simulink model "SIM_EXO_DAL"  (R2021b)
(part 14 of 25)

t5537 = t7.*t9.*t34.*t191.*t200.*2.245376163391997e-22;
t5541 = -t5527;
t5542 = t34.*t191.*t199.*1.213683123456844e-22;
t5543 = t8.*t19.*t34.*t191.*t201.*1.598755564896737e-22;
t5544 = t8.*t9.*t34.*t191.*t201.*8.501479316957259e-23;
t5548 = -t5534;
t5550 = t5.*t8.*t9.*t34.*t191.*t201.*2.432291264259161e-22;
t5551 = t5.*t34.*t191.*t200.*3.069039723904487e-29;
t5553 = t5.*t7.*t9.*t34.*t191.*t200.*4.590123554345229e-22;
t5554 = t7.*t19.*t34.*t191.*t200.*6.983254769046087e-22;
t5556 = t5.*t7.*t34.*t191.*t200.*1.220412967321392e-22;
t5567 = -t5559;
t5568 = t7.*t34.*t191.*t200.*3.484557373753613e-22;
t5570 = t5.*t7.*t34.*t191.*t199.*8.811397961779761e-29;
t5571 = t9.*t34.*t191.*t200.*4.024651742608185e-29;
t5572 = t8.*t34.*t191.*t201.*5.756958141897304e-23;
t5585 = t7.*t9.*t34.*t191.*t199.*1.155501764459885e-28;
t5587 = t34.*t191.*t200.*7.426504311526687e-22;
t5588 = t34.*t191.*t201.*7.426504311526687e-22;
t5595 = -t5594;
t5598 = t2449+t2464;
t5599 = t3.*t5597;
t5601 = (t615.*t4119)./2.0;
t5608 = t5.*t34.*t191.*t202.*7.477660125089319e-22;
t5609 = -t5606;
t5610 = t9.*t34.*t191.*t202.*4.064278195638759e-22;
t5613 = -t5611;
t5614 = t34.*t191.*t202.*5.900961483070041e-22;
t5616 = t633+t636+t1432;
t5620 = t635+t637+t1430;
t5621 = (t4.*t640.*t4119)./2.0;
t5631 = t34.*t191.*t201.*7.59040540289635e-22;
t5636 = t1492+t4150;
t5658 = t199+t2422+t2472;
t5659 = t3230+t3242;
t5663 = t3243+t3256;
t5664 = t3.*t5656;
t5665 = t7.*t5656;
t5669 = t4.*t5660;
t5670 = t8.*t5660;
t5778 = t656+t2601+t3257;
t5781 = t655+t2600+t3276;
t5796 = t2550+t5600;
t5812 = t1467+t5667;
t5815 = t1474+t5668;
t5825 = dq4.*t5823;
t5917 = (t4119.*t5779)./2.0;
t5958 = (t4119.*t5826)./2.0;
t5998 = (t4.*t4119.*t5887)./2.0;
t5999 = (t8.*t4119.*t5886)./2.0;
t7149 = dq3.*t7148;
t214 = -t208;
t217 = -t212;
t661 = t9.*t646;
t677 = t5.*t646;
t729 = -t691;
t803 = -t740;
t848 = t18.*t680;
t850 = t23.*t680;
t893 = -t844;
t894 = -t845;
t905 = -t856;
t907 = -t859;
t908 = -t858;
t912 = -t865;
t913 = -t866;
t915 = -t867;
t919 = -t876;
t931 = t18.*t799;
t932 = t8.*t847;
t938 = t23.*t799;
t985 = -t943;
t990 = -t947;
t998 = t8.*t909;
t1031 = -t963;
t1088 = -t1017;
t1090 = -t1021;
t1156 = -t1072;
t1201 = -t1135;
t1212 = -t1145;
t1213 = -t1149;
t1289 = -t1237;
t1292 = -t1241;
t1502 = -t1491;
t1516 = -t1500;
t1525 = -t1509;
t1544 = t5.*t1509;
t1546 = t9.*t1509;
t1600 = -t1564;
t1628 = -t1579;
t1655 = -t1601;
t1656 = -t1602;
t1707 = t8.*t1583;
t1708 = t8.*t1585;
t1732 = t18.*t1526;
t1742 = t23.*t1526;
t1762 = -t1686;
t1821 = -t1721;
t1860 = t8.*t1675;
t1863 = -t1747;
t1868 = -t1753;
t1870 = t8.*t1691;
t1878 = t8.*t1700;
t1899 = t8.*t1715;
t1901 = -t1794;
t1922 = t18.*t1577;
t1929 = t23.*t1577;
t1940 = -t1846;
t1941 = -t1845;
t1974 = t8.*t1765;
t1990 = t8.*t1777;
t2010 = -t1902;
t2034 = t8.*t1845;
t2039 = -t1934;
t2145 = -t2049;
t2233 = -t2161;
t2234 = -t2160;
t2242 = -t2164;
t2297 = -t2260;
t2298 = -t2259;
t2299 = -t2261;
t2300 = -t2262;
t2328 = -t2293;
t2330 = -t2301;
t2332 = -t2303;
t2354 = -t2320;
t2473 = -t2465;
t2670 = -t2632;
t2679 = -t2643;
t2690 = t5.*t2622;
t2691 = t5.*t2623;
t2696 = t9.*t2622;
t2697 = t9.*t2623;
t2698 = t5.*t2628;
t2700 = t9.*t2628;
t2701 = t5.*t2632;
t2704 = t9.*t2632;
t2709 = t5.*t2647;
t2710 = t5.*t2648;
t2711 = t5.*t2649;
t2712 = t9.*t2647;
t2713 = t9.*t2648;
t2714 = t9.*t2649;
t2715 = t5.*t2613;
t2718 = t9.*t2613;
t2727 = t5.*t2660;
t2728 = t5.*t2661;
t2730 = t9.*t2660;
t2731 = t9.*t2661;
t2732 = t5.*t2664;
t2735 = t9.*t2664;
t2777 = -t2745;
t2779 = t5.*t2689;
t2794 = t5.*t2740;
t2813 = t5.*t2750;
t2836 = -t2790;
t2850 = -t2811;
t2851 = -t2810;
t2858 = t9.*t2780;
t2873 = t9.*t2785;
t2880 = -t2838;
t2881 = -t2837;
t2887 = -t2841;
t2889 = -t2843;
t2890 = t9.*t2807;
t2905 = -t2860;
t2906 = -t2859;
t2909 = -t2865;
t2912 = -t2871;
t2913 = -t2870;
t2915 = -t2875;
t2916 = -t2874;
t2917 = -t2876;
t2933 = -t2891;
t2987 = -t2934;
t2998 = -t2955;
t2999 = -t2954;
t3000 = -t2957;
t3015 = -t2974;
t3125 = -t3102;
t3129 = -t3107;
t3159 = -t3135;
t3161 = -t3136;
t3164 = -t3138;
t3166 = -t3141;
t3168 = -t3144;
t3220 = -t3201;
t3221 = -t3203;
t3222 = -t3202;
t3223 = -t3205;
t3224 = -t3204;
t3237 = -t3214;
t3238 = -t3216;
t3239 = -t3215;
t3246 = -t3226;
t3248 = -t3227;
t3266 = -t3235;
t3268 = -t3249;
t3591 = -t3561;
t3621 = t9.*t3565;
t3627 = -t3594;
t3628 = -t3595;
t3665 = t5.*t3588;
t3672 = t9.*t3561;
t3673 = t5.*t3565;
t3675 = t5.*t3566;
t3683 = -t3623;
t3684 = -t3626;
t3689 = -t3632;
t3764 = t9.*t3632;
t3765 = t5.*t3640;
t3767 = -t3685;
t3771 = t9.*t3640;
t3799 = -t3731;
t3807 = -t3739;
t3808 = -t3740;
t3809 = -t3741;
t3829 = t5.*t3623;
t3830 = t5.*t3624;
t3838 = t5.*t3698;
t3841 = t9.*t3698;
t3842 = t5.*t3703;
t3844 = -t3775;
t3848 = t9.*t3703;
t3859 = -t3719;
t3864 = t5.*t3727;
t3874 = t9.*t3731;
t3876 = t5.*t3742;
t3878 = t9.*t3742;
t3879 = -t3801;
t3880 = -t3802;
t3896 = -t3828;
t3900 = t9.*t3775;
t3904 = t5.*t3779;
t3905 = -t3837;
t3906 = t5.*t3781;
t3907 = t9.*t3781;
t3909 = t9.*t3782;
t3919 = -t3791;
t3920 = -t3856;
t3926 = -t3860;
t3927 = -t3861;
t3933 = t9.*t3801;
t3936 = t9.*t3802;
t3940 = t5.*t3812;
t3943 = t5.*t3818;
t3944 = t9.*t3818;
t3948 = -t3887;
t3955 = -t3902;
t3956 = -t3901;
t3957 = -t3903;
t3961 = t9.*t3856;
t3965 = t5.*t3865;
t3967 = t5.*t3868;
t3969 = t9.*t3868;
t3973 = -t3932;
t3975 = -t3935;
t3976 = -t3934;
t3977 = -t3938;
t3978 = -t3937;
t3979 = -t3939;
C_dq = ft_11({dq1,dq2,dq3,dq4,dq5,dq6,t1004,t1006,t1008,t1013,t1016,t1019,t1020,t1023,t1024,t1025,t1026,t1028,t1030,t1031,t1032,t1034,t1036,t1038,t1039,t1040,t1042,t1043,t1044,t1045,t1046,t1047,t1048,t1049,t1050,t1051,t1054,t1055,t1056,t1057,t1059,t1061,t1065,t1066,t1068,t1069,t1070,t1073,t1075,t1076,t1077,t1081,t1083,t1084,t1085,t1087,t1088,t1089,t1090,t1091,t1092,t1093,t1095,t1098,t1099,t1101,t1102,t1105,t1106,t1107,t1108,t1109,t111,t1113,t1115,t1116,t1119,t112,t1122,t1125,t1126,t1127,t1128,t113,t1130,t1131,t1133,t1134,t1138,t1139,t114,t1141,t1144,t1146,t1147,t1148,t115,t1150,t1152,t1153,t1155,t1156,t1158,t1159,t116,t1162,t1163,t1165,t1167,t1169,t1170,t1171,t1173,t1174,t1175,t1177,t1178,t1179,t1180,t1181,t1182,t1183,t1184,t1185,t1186,t1188,t1189,t1190,t1191,t1192,t1193,t1194,t1196,t1197,t1198,t1199,t1200,t1201,t1202,t1203,t1204,t1205,t1206,t1207,t121,t1210,t1211,t1212,t1213,t1215,t1219,t1221,t1222,t1224,t1225,t1227,t1228,t1233,t1235,t1236,t1239,t1240,t1244,t1245,t125,t1250,t1251,t1253,t1254,t1256,t1257,t1258,t1259,t126,t1261,t1262,t1263,t1264,t1265,t1266,t1267,t1268,t1269,t1271,t1272,t1273,t1274,t1277,t1278,t128,t1280,t1282,t1285,t1286,t1288,t1289,t1290,t1292,t1294,t1295,t1296,t1298,t1300,t1301,t1302,t1306,t1307,t1308,t1309,t131,t1311,t1312,t1313,t1315,t1316,t1317,t1318,t1319,t132,t1322,t1323,t1324,t1325,t1326,t1328,t1329,t133,t1330,t1331,t1333,t1337,t1338,t1340,t1341,t1342,t1343,t1344,t1345,t1346,t1348,t1351,t1352,t1353,t1354,t1355,t1356,t1360,t1362,t1365,t1366,t1367,t1369,t1370,t1371,t1372,t1374,t1375,t1377,t1378,t1379,t1380,t1383,t1384,t1385,t1386,t1388,t1389,t139,t1391,t1392,t1393,t1394,t1397,t140,t1401,t1402,t1403,t1404,t1406,t1407,t1408,t1409,t141,t1410,t1411,t1413,t1414,t1415,t1416,t1417,t1419,t142,t1423,t1426,t1427,t1428,t1429,t1431,t1433,t1436,t144,t1440,t1441,t1442,t1443,t1445,t1446,t1447,t1448,t1449,t1451,t1452,t1453,t1454,t1455,t1456,t1457,t1458,t1459,t1460,t1463,t1464,t1465,t1470,t1471,t1476,t1478,t1479,t148,t1481,t1482,t1483,t1486,t1487,t1488,t1489,t1490,t1493,t1494,t1495,t1496,t1498,t1499,t15,t150,t1501,t1502,t1503,t1505,t1506,t1507,t1508,t151,t1510,t1511,t1512,t1513,t1515,t1516,t1517,t1520,t1521,t1522,t1523,t1524,t1525,t1526,t1527,t1529,t153,t1530,t1531,t1532,t1533,t1534,t1535,t1536,t1537,t1538,t1539,t154,t1540,t1541,t1542,t1546,t1548,t1549,t1550,t1551,t1553,t1558,t156,t1560,t1561,t1562,t1566,t1567,t1568,t1570,t1571,t1572,t1574,t1575,t1576,t1577,t1578,t158,t1580,t1581,t1582,t1583,t1584,t1585,t1586,t1587,t1589,t1590,t1591,t1592,t1593,t1594,t1595,t1596,t1597,t1598,t1599,t16,t1600,t1601,t1602,t1605,t1606,t1607,t1609,t1610,t1611,t1612,t1613,t1614,t1615,t1616,t1617,t1618,t1619,t1620,t1621,t1622,t1625,t1626,t1627,t1628,t1630,t1631,t1632,t1633,t1635,t1636,t1637,t1638,t1639,t1641,t1642,t1643,t1644,t1645,t1646,t1647,t1648,t1651,t1652,t1653,t1655,t1656,t1657,t1658,t1659,t166,t1660,t1661,t1662,t1663,t1666,t1667,t1669,t1670,t1671,t1672,t1673,t1674,t1675,t1676,t1681,t1682,t1683,t1687,t1689,t1692,t1696,t1697,t1698,t1699,t17,t1700,t1701,t1702,t1703,t1704,t1705,t1706,t1707,t1708,t1709,t171,t1710,t1711,t1712,t1713,t1715,t1716,t1718,t1719,t1720,t1721,t1722,t1723,t1724,t1726,t1728,t1729,t1731,t1732,t1733,t1734,t1735,t1736,t1737,t1738,t1739,t1740,t1741,t1742,t1745,t1746,t1747,t1748,t1749,t1752,t1753,t1754,t1755,t1756,t1757,t1758,t1759,t1760,t1761,t1762,t1763,t1764,t1765,t1766,t1767,t1768,t1769,t1770,t1771,t1772,t1774,t1775,t1776,t1777,t1779,t1780,t1781,t1783,t1784,t1785,t1786,t1787,t1788,t1789,t1790,t1791,t1792,t1793,t1794,t1795,t1797,t1798,t1799,t18,t1800,t1801,t1804,t1805,t1806,t1807,t1808,t1809,t1810,t1811,t1812,t1813,t1814,t1815,t1816,t1817,t1820,t1821,t1822,t1823,t1824,t1827,t1828,t1829,t183,t1830,t1831,t1832,t1833,t1834,t1835,t1836,t1837,t1838,t1839,t1844,t1847,t1848,t1849,t185,t1850,t1851,t1853,t1855,t1856,t1857,t1858,t1859,t1860,t1861,t1863,t1864,t1865,t1866,t1867,t1868,t1870,t1871,t1873,t1877,t1878,t1879,t1881,t1882,t1884,t1885,t1886,t1887,t1889,t1891,t1892,t1893,t1896,t1899,t19,t190,t1900,t1901,t1902,t1903,t1905,t1906,t1907,t1908,t1909,t191,t1910,t1911,t1912,t1913,t1914,t1915,t1916,t1917,t1918,t1919,t1920,t1921,t1922,t1925,t1926,t1927,t1928,t1929,t1930,t1935,t1936,t1937,t1938,t1939,t1940,t1941,t1942,t1943,t1944,t1946,t1947,t1950,t1951,t1952,t1953,t1954,t1955,t196,t1961,t1966,t1967,t1968,t1969,t197,t1970,t1971,t1974,t1975,t1976,t1977,t1978,t1979,t1980,t1981,t1983,t1984,t1985,t1986,t1987,t1988,t1989,t199,t1990,t1991,t1992,t1993,t1994,t1995,t1996,t1997,t1998,t1999,t2,t20,t200,t2000,t2001,t2002,t2003,t2004,t2005,t2006,t2008,t201,t2010,t2011,t2014,t2015,t2016,t2017,t2018,t2019,t202,t2020,t2023,t2024,t2026,t2027,t2028,t2029,t203,t2033,t2034,t2035,t2036,t2037,t2038,t2039,t204,t2040,t2042,t2043,t2045,t2047,t205,t2050,t2051,t2052,t2053,t2054,t2056,t2057,t2058,t2059,t206,t2060,t2061,t2062,t2065,t2066,t2067,t2068,t2069,t207,t2070,t2071,t2072,t2073,t2074,t2075,t2076,t2077,t2078,t2079,t2081,t2082,t2083,t2084,t2085,t2086,t2087,t2088,t2089,t209,t2090,t2091,t2092,t2093,t2094,t2095,t2096,t2097,t2098,t2099,t21,t210,t2100,t2101,t2104,t2105,t2106,t2107,t2108,t2109,t211,t2110,t2111,t2113,t2114,t2115,t2116,t2117,t2118,t2119,t2121,t2123,t2125,t2127,t2128,t2129,t213,t2130,t2131,t2132,t2133,t2134,t2135,t2136,t2137,t2138,t214,t2142,t2143,t2144,t2145,t2146,t2148,t2149,t2150,t2151,t2152,t2154,t2155,t2156,t2157,t2158,t2159,t2164,t2165,t2166,t2169,t217,t2170,t2171,t2172,t2174,t2175,t2176,t2177,t2178,t2180,t2181,t2182,t2184,t2185,t2186,t2187,t2189,t2190,t2191,t2192,t2193,t2194,t2196,t2197,t2198,t2199,t22,t2200,t2201,t2202,t2203,t2204,t2208,t2209,t2211,t2212,t2213,t2214,t2215,t2216,t2217,t2218,t2219,t2220,t2221,t2223,t2224,t2225,t2227,t2228,t2229,t2230,t2231,t2232,t2233,t2234,t2236,t2237,t2238,t2239,t224,t2240,t2241,t2242,t2243,t2246,t2247,t2248,t2249,t225,t2251,t2253,t2254,t2256,t2257,t2258,t2263,t2264,t2265,t2266,t2267,t2268,t2269,t227,t2270,t2271,t2272,t2273,t2274,t2276,t2277,t2278,t2279,t228,t2280,t2281,t2282,t2283,t2284,t2285,t2286,t2288,t2289,t2290,t2291,t2295,t2296,t2297,t2298,t2299,t23,t230,t2300,t2302,t2303,t2304,t2305,t2306,t2307,t2308,t231,t2310,t2311,t2312,t2313,t2314,t2315,t2316,t2317,t2318,t2319,t2320,t2321,t2322,t2323,t2324,t2326,t2327,t2328,t233,t2330,t2331,t2332,t2333,t2334,t2336,t2337,t2338,t2339,t234,t2340,t2341,t2342,t2344,t2345,t2346,t2347,t2348,t235,t2350,t2354,t2355,t2357,t2358,t2359,t236,t2361,t2362,t2363,t2364,t2365,t2366,t2367,t2369,t2370,t2371,t2372,t2373,t2374,t2375,t2376,t2377,t2378,t2379,t2382,t2383,t2384,t2385,t2386,t2387,t2388,t2389,t2390,t2391,t2392,t2393,t2394,t2395,t2396,t2397,t2398,t24,t240,t2400,t2401,t2402,t2403,t2404,t2405,t2406,t2407,t2408,t2410,t2416,t2417,t2420,t2421,t2422,t2424,t2425,t2426,t2427,t2428,t2429,t243,t2430,t2431,t2434,t2435,t2437,t2438,t2439,t244,t2440,t2441,t2443,t2444,t2446,t2448,t2449,t2452,t2453,t2454,t2455,t2456,t2457,t2458,t2460,t2463,t2465,t2466,t2467,t2470,t2473,t2474,t2477,t2478,t2479,t2481,t2483,t2484,t2485,t2486,t2487,t2489,t249,t2490,t2494,t2495,t2497,t2500,t2502,t2503,t2505,t2507,t2508,t2510,t2511,t2512,t2513,t2517,t2518,t2519,t2520,t2521,t2522,t2523,t2524,t2525,t2526,t2527,t2530,t2531,t2533,t2534,t2535,t2536,t2537,t2539,t2540,t2541,t2542,t2543,t2544,t2545,t2546,t2547,t2548,t2549,t2552,t2553,t2554,t2555,t2556,t2560,t2562,t2563,t2564,t2565,t2566,t2567,t2568,t2569,t257,t2570,t2571,t2574,t2575,t2576,t2577,t2578,t2579,t258,t2581,t2582,t2585,t2586,t2587,t2588,t2589,t2590,t2594,t2595,t2597,t2598,t2599,t2602,t2603,t2604,t2606,t2607,t2608,t2611,t2612,t2613,t2614,t2615,t2616,t2617,t2620,t2622,t2623,t2624,t2625,t2626,t2627,t2628,t2629,t263,t2630,t2631,t2633,t2634,t2636,t2639,t2640,t2641,t2644,t2647,t2648,t2649,t2650,t2651,t2654,t2655,t2656,t2657,t2659,t266,t2660,t2661,t2662,t2663,t2664,t2665,t2666,t2668,t2669,t2670,t2671,t2673,t2675,t2676,t2677,t2678,t2679,t2680,t2681,t2682,t2684,t2685,t2686,t2688,t2689,t2691,t2692,t2693,t2694,t2695,t2696,t2697,t2698,t2699,t270,t2700,t2701,t2705,t2706,t2707,t2708,t2711,t2712,t2713,t2714,t2715,t2718,t2719,t2720,t2721,t2722,t2723,t2724,t2725,t2726,t2728,t2729,t273,t2730,t2731,t2732,t2735,t2736,t2737,t2738,t274,t2740,t2741,t2742,t2743,t2744,t2746,t2747,t2748,t2749,t275,t2750,t2752,t2753,t2754,t2755,t2756,t2757,t2758,t2759,t276,t2760,t2761,t2762,t2763,t2764,t2765,t2766,t2767,t2769,t277,t2770,t2771,t2772,t2774,t2775,t2777,t2778,t278,t2780,t2783,t2784,t2785,t2791,t2792,t2793,t2795,t2796,t2797,t2798,t2799,t280,t2800,t2801,t2802,t2803,t2805,t2806,t2807,t2809,t2812,t2814,t2815,t2816,t2817,t2818,t2819,t2820,t2822,t2823,t2824,t2825,t2826,t2827,t2828,t2829,t2830,t2831,t2832,t2833,t2834,t2835,t2836,t2839,t284,t2842,t2844,t2845,t2846,t2850,t2851,t2852,t2854,t2857,t2861,t2863,t2864,t2867,t2868,t2869,t287,t2872,t2877,t2878,t2880,t2881,t2882,t2883,t2884,t2885,t2886,t2887,t2888,t2889,t2892,t2893,t2894,t2895,t2896,t2897,t29,t290,t2900,t2903,t2904,t2905,t2906,t2907,t2908,t2909,t291,t2910,t2911,t2912,t2913,t2914,t2915,t2916,t2917,t2918,t2919,t292,t2920,t2921,t2922,t2923,t2925,t2928,t2929,t2930,t2931,t2932,t2933,t2937,t294,t2940,t2941,t2942,t2944,t2945,t2946,t2947,t2949,t2950,t2951,t2952,t2956,t2958,t2959,t2962,t2965,t2966,t2967,t2968,t2969,t297,t2970,t2971,t2972,t2973,t2975,t2977,t2978,t2980,t2983,t2984,t2985,t2986,t2987,t2988,t2989,t299,t2991,t2992,t2993,t2994,t2995,t2996,t2997,t2998,t2999,t3,t30,t300,t3000,t3001,t3002,t3003,t3005,t3007,t3008,t3010,t3011,t3013,t3014,t3015,t3018,t3019,t302,t3020,t3021,t3022,t3024,t3025,t3027,t3029,t303,t3030,t3031,t3032,t3033,t3034,t3035,t3036,t3037,t3038,t304,t3041,t3043,t3044,t3046,t3047,t3048,t3049,t305,t3050,t3051,t3052,t3053,t3054,t3055,t3056,t3057,t3059,t306,t3060,t3061,t3062,t3064,t3065,t3066,t3067,t3068,t3069,t3070,t3071,t3072,t3073,t3074,t3076,t3077,t3079,t3080,t3081,t3082,t3083,t3084,t3085,t3086,t3088,t3089,t309,t3090,t3092,t3094,t3095,t3096,t3097,t3098,t3099,t310,t3100,t3103,t3104,t3105,t3106,t3108,t3109,t311,t3110,t3112,t3113,t3114,t3117,t3118,t3119,t3120,t3121,t3122,t3123,t3124,t3125,t3126,t3127,t3128,t3129,t313,t3130,t3131,t3132,t3133,t3134,t3136,t3139,t314,t3140,t3142,t3143,t3146,t3148,t3149,t315,t3150,t3152,t3153,t3154,t3156,t3157,t3158,t3159,t316,t3160,t3161,t3163,t3164,t3166,t3167,t3168,t3169,t3170,t3171,t3172,t3174,t3175,t3176,t3178,t3179,t318,t3180,t3182,t3183,t3184,t3185,t3186,t3187,t3188,t3189,t319,t3190,t3191,t3192,t3193,t3194,t3195,t3196,t3198,t3199,t320,t3200,t3207,t3208,t3209,t3210,t3213,t3217,t3219,t322,t3220,t3221,t3222,t3223,t3224,t3228,t3229,t3230,t3232,t3234,t3236,t3237,t3238,t3239,t324,t3240,t3245,t3246,t3247,t3248,t325,t3250,t3251,t3252,t3254,t3265,t3266,t3267,t3268,t3269,t3270,t3271,t3272,t3273,t3274,t3275,t3277,t3278,t3279,t328,t3280,t3282,t3283,t3284,t3285,t3286,t3287,t3288,t3289,t3290,t3291,t3292,t3293,t3295,t3296,t3297,t3298,t3299,t3301,t3302,t3303,t3306,t3307,t3308,t3309,t3310,t3312,t3313,t3314,t3317,t3318,t3320,t3321,t3322,t3323,t3324,t3325,t3326,t3327,t3328,t3329,t333,t3331,t3332,t3333,t3334,t3335,t3336,t3337,t3338,t3339,t3340,t3341,t3342,t3343,t3346,t3347,t3349,t3350,t3351,t3352,t3353,t3354,t3356,t3357,t3358,t3359,t336,t3360,t3362,t3363,t3364,t3365,t3366,t3367,t3368,t3369,t337,t3371,t3372,t3373,t3374,t3375,t3376,t3377,t3378,t3380,t3381,t3382,t3383,t3384,t3386,t3387,t3388,t3390,t3391,t3392,t3393,t3394,t3395,t3396,t3397,t3398,t3399,t34,t340,t3400,t3402,t3403,t3404,t3405,t3407,t3408,t3409,t3410,t3411,t3412,t3413,t3416,t3417,t3418,t3420,t3421,t3422,t3423,t3424,t3425,t3426,t3427,t3429,t3430,t3431,t3432,t3433,t3434,t3435,t3436,t3437,t3439,t344,t3440,t3441,t3442,t3443,t3444,t3445,t3446,t3447,t3448,t3449,t3450,t3453,t3454,t3455,t3456,t3457,t3458,t346,t3460,t3461,t3462,t3463,t3464,t3465,t3466,t3467,t3468,t3469,t347,t3470,t3471,t3472,t3473,t3474,t3475,t3476,t3479,t348,t3480,t3481,t3483,t3484,t3485,t3487,t3488,t3489,t349,t3490,t3491,t3492,t3493,t3494,t3496,t3497,t3498,t3499,t350,t3500,t3501,t3502,t3503,t3504,t3505,t3506,t3507,t3509,t3510,t3511,t3513,t3514,t3515,t3516,t3517,t3518,t352,t3521,t3522,t3523,t3526,t3529,t353,t3530,t3531,t3532,t3533,t3535,t3536,t3538,t3539,t3540,t3542,t3543,t3544,t3546,t3547,t3549,t3551,t3552,t3554,t3556,t3557,t3559,t356,t3560,t3562,t3563,t3564,t3565,t3566,t3568,t3569,t357,t3570,t3571,t3572,t3573,t3574,t3577,t3578,t358,t3582,t3583,t3584,t3585,t3586,t3587,t3588,t3589,t359,t3590,t3591,t3592,t3593,t3595,t3596,t3597,t3598,t3599,t3600,t3602,t3603,t3604,t3605,t3606,t3607,t3609,t361,t3610,t3611,t3612,t3616,t3617,t3618,t362,t3624,t3625,t3627,t3628,t3630,t3631,t3633,t3634,t3635,t3636,t3637,t3638,t3640,t3642,t3644,t3648,t365,t3652,t3653,t3654,t3655,t3656,t3657,t3658,t3659,t3660,t3662,t3663,t3664,t3665,t3666,t3667,t3668,t3669,t3670,t3671,t3672,t3673,t3674,t3675,t3676,t3677,t3678,t3679,t368,t3681,t3682,t3683,t3684,t3687,t3689,t369,t3690,t3691,t3692,t3693,t3694,t3695,t3696,t3697,t3698,t3699,t3700,t3701,t3702,t3703,t3704,t3705,t3706,t3707,t3708,t3709,t371,t3711,t3712,t3713,t3715,t3716,t3717,t3718,t3719,t372,t3720,t3724,t3725,t3726,t3727,t3728,t3729,t373,t3730,t3731,t3732,t3733,t3734,t3735,t3736,t3737,t3738,t374,t3740,t3742,t3743,t3744,t3745,t3746,t3747,t3750,t3752,t3753,t3754,t3755,t3756,t3757,t3758,t3759,t3760,t3761,t3762,t3763,t3764,t3765,t3766,t3767,t3768,t3769,t377,t3772,t3774,t3777,t3778,t3779,t378,t3780,t3781,t3782,t3783,t3784,t3785,t3786,t3787,t3788,t3789,t379,t3790,t3791,t3792,t3793,t3794,t3795,t3796,t3797,t3798,t3799,t380,t3800,t3807,t3808,t3809,t3810,t3811,t3812,t3813,t3814,t3815,t3816,t3817,t3818,t3819,t382,t3820,t3821,t3822,t3823,t3824,t3825,t3830,t3831,t3833,t3834,t3835,t3836,t3838,t3839,t384,t3840,t3841,t3842,t3843,t3844,t3845,t3848,t3849,t3850,t3851,t3852,t3853,t3855,t3859,t386,t3861,t3862,t3863,t3864,t3865,t3866,t3868,t3869,t387,t3870,t3871,t3872,t3873,t3874,t3875,t3876,t3877,t3879,t388,t3880,t3881,t3882,t3883,t3884,t3885,t3886,t3888,t3889,t3890,t3891,t3892,t3893,t3894,t3895,t3896,t3897,t3899,t3900,t3904,t3905,t3906,t3907,t3908,t3909,t391,t3910,t3911,t3912,t3913,t3914,t3915,t3916,t3917,t3918,t3919,t392,t3920,t3921,t3922,t3923,t3924,t3925,t3926,t3927,t3928,t3931,t3936,t3940,t3941,t3942,t3943,t3944,t3946,t3948,t395,t3950,t3951,t3952,t3953,t3954,t3955,t3956,t3957,t3958,t3959,t396,t3960,t3961,t3962,t3963,t3964,t3965,t3966,t3967,t3968,t3969,t3971,t3972,t3973,t3974,t3975,t3976,t3977,t3978,t3979,t3982,t3983,t3984,t3985,t3986,t3987,t3988,t3989,t3994,t3995,t3996,t3997,t4,t400,t4000,t4003,t4004,t4006,t4008,t4009,t401,t4010,t4011,t4012,t4013,t4014,t4015,t4016,t4017,t4018,t4019,t402,t4020,t4022,t4023,t4024,t4025,t4026,t4028,t4029,t403,t4034,t4035,t4037,t4038,t4039,t4040,t4041,t4042,t4045,t4046,t4047,t4048,t4049,t4050,t4051,t4053,t4054,t4055,t4056,t4057,t4059,t406,t4060,t4061,t4062,t4063,t4064,t4065,t4066,t4067,t4068,t4069,t4070,t4071,t4073,t4074,t4075,t4079,t4080,t4081,t4082,t4083,t4084,t4085,t4086,t4087,t4089,t4090,t4091,t4092,t4093,t4094,t4095,t4097,t4098,t4099,t410,t4100,t4103,t4105,t4106,t4108,t4109,t411,t4110,t4111,t4112,t4113,t4114,t4115,t4116,t4118,t4119,t412,t4120,t4123,t4124,t4125,t4126,t4127,t4128,t4129,t413,t4130,t4132,t4133,t4134,t4135,t4136,t4139,t414,t4140,t4141,t4142,t4143,t4144,t4145,t4147,t4148,t4149,t415,t4151,t4152,t4153,t4154,t416,t4161,t4162,t4164,t4165,t4166,t4169,t417,t4171,t4173,t4174,t4177,t4178,t4179,t418,t4180,t4181,t4183,t4184,t4185,t4186,t4188,t4190,t4195,t4196,t4197,t420,t4201,t4202,t4205,t4206,t4207,t4208,t4209,t4210,t4211,t4215,t4217,t4218,t4219,t422,t4220,t4221,t4223,t4224,t4225,t4226,t4228,t4229,t423,t4230,t4231,t4232,t4233,t4234,t4235,t424,t4241,t4242,t4243,t4244,t4245,t4246,t4247,t4248,t4249,t425,t4250,t4251,t4253,t4254,t4255,t4256,t4257,t4258,t4259,t4260,t4261,t4262,t4263,t427,t4273,t4274,t4275,t4276,t4278,t4279,t428,t4280,t4281,t4282,t4283,t4284,t4285,t4286,t4287,t4289,t429,t4290,t4291,t4292,t4293,t4295,t4296,t4297,t4298,t4299,t4300,t4301,t4302,t4303,t4304,t4305,t4306,t4308,t431,t4310,t4315,t4316,t4317,t4318,t432,t4321,t4323,t4324,t4325,t4326,t4327,t4328,t4329,t433,t4330,t4331,t4332,t4333,t4334,t4335,t4336,t4337,t4338,t4339,t434,t4340,t4342,t4344,t4345,t4346,t4347,t4348,t4349,t435,t4350,t4354,t4356,t4357,t436,t4362,t4363,t4365,t4366,t4368,t4369,t437,t4370,t4371,t4372,t4373,t4374,t4375,t4376,t4377,t4378,t4379,t438,t4380,t4382,t4383,t4384,t4385,t4386,t4387,t4388,t4389,t439,t4391,t4392,t4394,t4395,t4396,t4397,t4398,t4399,t44,t440,t4400,t4401,t4402,t4403,t4404,t4405,t4406,t4407,t4408,t4409,t441,t4410,t4411,t4412,t4413,t4414,t4415,t4416,t4417,t4418,t4419,t442,t4420,t4421,t4422,t4423,t4424,t4425,t4426,t4427,t4428,t4429,t4430,t4431,t4432,t4433,t4434,t4435,t4436,t4437,t4438,t4439,t444,t4440,t4442,t4444,t4445,t4446,t4447,t4448,t4449,t445,t4450,t4451,t4453,t4454,t4455,t4460,t4461,t4462,t4463,t4464,t4465,t4466,t4467,t4468,t4469,t4470,t4471,t4473,t4474,t4475,t4476,t4477,t4478,t4479,t448,t4481,t4482,t4483,t4484,t4485,t4486,t4487,t4488,t4489,t449,t4490,t4493,t4494,t4495,t4496,t4497,t4498,t4499,t45,t450,t4500,t4501,t4502,t4503,t4504,t4505,t4506,t4507,t4508,t4509,t4510,t4512,t4513,t4514,t4515,t4516,t4518,t4519,t452,t4520,t4521,t4522,t4523,t4524,t4525,t4526,t4527,t4529,t453,t4530,t4531,t4532,t4534,t4535,t4536,t4537,t4538,t4539,t454,t4541,t4543,t4544,t4545,t4546,t4547,t4549,t4550,t4551,t4552,t4553,t4554,t4556,t4557,t4558,t4559,t4560,t4564,t4565,t4566,t4567,t4568,t4569,t457,t4570,t4572,t4573,t4575,t4576,t4577,t4578,t458,t4580,t4581,t4582,t4584,t4585,t4586,t4587,t4588,t4589,t459,t4590,t4591,t4592,t4593,t4594,t4595,t4596,t4597,t4598,t4599,t46,t460,t4600,t4601,t4602,t4603,t4604,t4605,t4606,t4607,t4608,t4609,t461,t4610,t4612,t4613,t4614,t4615,t4616,t4617,t4618,t4619,t462,t4620,t4621,t4622,t4623,t4624,t4625,t4626,t4627,t4629,t463,t4631,t4632,t4633,t4634,t4635,t4636,t4637,t4638,t4639,t464,t4640,t4643,t4644,t4645,t4646,t4647,t4648,t4649,t465,t4650,t4652,t4653,t4654,t4655,t4656,t4657,t4659,t466,t4660,t4661,t4662,t4663,t4664,t4665,t4666,t4667,t4668,t4669,t4670,t4671,t4672,t4673,t4674,t4675,t4676,t4677,t4678,t4679,t468,t4680,t4681,t4682,t4683,t4684,t4685,t4686,t4687,t4689,t469,t4692,t4693,t4694,t4695,t4696,t4697,t4698,t4699,t47,t470,t4700,t4702,t4703,t4704,t4707,t4708,t4709,t471,t4710,t4711,t4712,t4713,t4714,t4715,t4716,t4717,t4718,t4719,t472,t4720,t4721,t4722,t4723,t4724,t4725,t4726,t4727,t4728,t4729,t4730,t4731,t4732,t4733,t4734,t4736,t4737,t4738,t4739,t4740,t4742,t4745,t4746,t4747,t4748,t475,t4750,t4751,t4753,t4754,t4755,t4756,t4757,t4762,t4763,t4765,t4768,t477,t4771,t4772,t4773,t4774,t4775,t4776,t4779,t4780,t4781,t4782,t4783,t4784,t4785,t4786,t4787,t4788,t4789,t479,t4790,t4791,t4792,t4793,t4794,t4795,t4797,t4799,t480,t4800,t4801,t4802,t4803,t4805,t4806,t4809,t481,t4810,t4811,t4812,t4813,t4814,t4816,t4817,t4818,t4819,t482,t4820,t4822,t4823,t4824,t4825,t4826,t4827,t4829,t483,t4831,t4833,t4834,t4835,t4837,t484,t4840,t4841,t4842,t4843,t4844,t4845,t4846,t4848,t485,t4850,t4853,t4854,t4855,t4856,t4857,t4858,t4859,t486,t4862,t4863,t4864,t4865,t4866,t4867,t4868,t4869,t4870,t4872,t4873,t4874,t4875,t4876,t4877,t488,t4880,t4881,t4884,t4888,t4889,t489,t4890,t4893,t4894,t4895,t4896,t4898,t4901,t4902,t4903,t4904,t4905,t4906,t4907,t4908,t491,t4911,t4913,t4914,t4919,t492,t4920,t4922,t4924,t4925,t4927,t4928,t4929,t493,t4931,t4932,t4933,t4934,t4935,t4936,t4939,t494,t4942,t4943,t4944,t4946,t4947,t4948,t4949,t4950,t4951,t4952,t4953,t4957,t4959,t496,t4960,t4961,t4963,t4964,t4965,t4966,t4967,t4969,t497,t4970,t4973,t4974,t4975,t4976,t4978,t4979,t498,t4981,t4982,t4983,t4984,t4987,t4988,t4989,t499,t4990,t4991,t4992,t4993,t4994,t4995,t4996,t5,t50,t500,t5000,t5001,t5002,t5003,t5005,t5006,t5007,t5008,t5009,t501,t5010,t5013,t5014,t5015,t5016,t5017,t5018,t5019,t502,t5020,t5021,t5022,t5023,t5024,t5026,t5027,t5028,t5029,t503,t5031,t5032,t5035,t5036,t5037,t5039,t504,t5041,t5045,t5047,t5048,t505,t5051,t5054,t5055,t5056,t5057,t5058,t5059,t506,t5061,t5063,t5064,t5065,t5066,t5067,t5068,t507,t5073,t5074,t5075,t5076,t5077,t5078,t5079,t508,t5080,t5083,t5084,t5085,t5086,t5087,t5088,t5089,t509,t5090,t5091,t5092,t5093,t5094,t5095,t5097,t5098,t5099,t510,t5100,t5101,t5102,t5103,t5104,t5105,t5107,t5109,t511,t5110,t5112,t5113,t5114,t5117,t5118,t5119,t512,t5120,t5121,t5123,t5124,t5126,t5128,t513,t5131,t5132,t5133,t5134,t5135,t5136,t5137,t5138,t5139,t514,t5140,t5141,t5143,t5146,t5147,t5148,t5150,t5151,t5154,t5156,t5157,t5158,t5159,t516,t5160,t5162,t5164,t5166,t5167,t517,t5171,t5172,t5173,t5174,t5175,t5177,t518,t5180,t5181,t5182,t5183,t5184,t5185,t5187,t5188,t5189,t5190,t5191,t5194,t5195,t5197,t5199,t520,t5200,t5201,t5202,t5203,t5204,t5205,t5206,t5207,t5209,t521,t5210,t5211,t5213,t5214,t5215,t5216,t5217,t5218,t5219,t522,t5220,t5221,t5222,t5223,t5224,t5225,t5226,t5227,t5229,t523,t5233,t5236,t5237,t5238,t5239,t524,t5240,t5242,t5243,t5244,t5247,t5248,t5249,t525,t5251,t5252,t5255,t5258,t526,t5261,t5262,t5265,t5268,t5269,t527,t5270,t5272,t5275,t5276,t5277,t5278,t5279,t528,t5280,t5285,t5287,t5288,t529,t5291,t5292,t5293,t5294,t5295,t5297,t5298,t53,t530,t5302,t5303,t5304,t5306,t5308,t531,t5310,t5317,t5318,t532,t5320,t5321,t5322,t5324,t5326,t5327,t5329,t533,t5330,t5331,t5332,t5334,t5336,t5339,t534,t5341,t5344,t5346,t5347,t5348,t5349,t535,t5351,t5355,t5356,t5358,t5359,t536,t5361,t5364,t5365,t5367,t5368,t537,t5372,t5373,t5374,t5375,t5378,t538,t5383,t5386,t5387,t5388,t5389,t539,t5390,t5391,t5392,t5393,t5394,t5395,t540,t5402,t5404,t5406,t5408,t5409,t5411,t5416,t5420,t543,t5433,t5435,t5436,t5437,t5438,t544,t5440,t5441,t5442,t5443,t5444,t5445,t5448,t545,t5450,t5451,t5453,t5454,t5457,t5459,t546,t5460,t5461,t5462,t5463,t5464,t5465,t5466,t547,t5473,t5475,t5479,t548,t5480,t5481,t5482,t5483,t5484,t5485,t5486,t5487,t5488,t5489,t549,t5490,t5491,t5492,t5493,t5494,t5495,t5498,t5499,t5500,t5501,t5502,t5503,t5504,t5505,t5506,t5507,t551,t5512,t5513,t5514,t5516,t5517,t5518,t5519,t552,t5520,t5521,t5523,t5524,t5525,t5526,t5528,t553,t5531,t5533,t5536,t5537,t554,t5540,t5541,t5542,t5543,t5544,t5546,t5548,t5549,t555,t5550,t5551,t5552,t5553,t5554,t5555,t5556,t556,t5561,t5562,t5563,t5565,t5566,t5567,t5568,t5569,t557,t5570,t5571,t5572,t5573,t5578,t558,t5580,t5581,t5583,t5584,t5585,t5587,t5588,t5589,t559,t5590,t5593,t5595,t5596,t5599,t560,t5601,t5603,t5604,t5607,t5608,t5609,t561,t5610,t5612,t5613,t5614,t5616,t5618,t562,t5620,t5621,t5629,t563,t5631,t5633,t5634,t5635,t5636,t564,t5658,t5664,t5665,t5669,t567,t5670,t5673,t5678,t568,t5688,t569,t57,t570,t571,t572,t573,t574,t5741,t5743,t576,t577,t5777,t5778,t5779,t578,t5780,t5781,t5782,t579,t58,t580,t581,t5815,t5818,t5819,t582,t5823,t5825,t5826,t583,t584,t586,t587,t5886,t5887,t589,t5894,t59,t590,t591,t5917,t592,t593,t594,t595,t5958,t596,t597,t5998,t5999,t6,t60,t600,t602,t603,t604,t605,t609,t610,t611,t612,t613,t614,t615,t616,t618,t619,t620,t621,t622,t623,t624,t625,t626,t629,t632,t633,t634,t638,t639,t640,t641,t642,t643,t645,t646,t647,t648,t649,t650,t653,t654,t657,t658,t660,t661,t662,t663,t664,t665,t667,t668,t669,t673,t674,t675,t676,t677,t679,t680,t681,t682,t683,t684,t685,t686,t687,t688,t689,t692,t693,t694,t695,t696,t697,t698,t7,t700,t702,t703,t704,t705,t706,t708,t71,t710,t711,t712,t713,t7148,t7149,t715,t716,t72,t724,t728,t729,t73,t731,t733,t734,t735,t736,t738,t739,t74,t741,t742,t743,t744,t746,t747,t748,t749,t75,t750,t751,t752,t753,t754,t755,t756,t757,t758,t759,t76,t760,t762,t763,t764,t765,t766,t767,t768,t769,t77,t772,t773,t774,t775,t776,t777,t778,t779,t780,t781,t782,t784,t785,t786,t792,t794,t795,t796,t797,t798,t799,t8,t80,t801,t802,t803,t804,t805,t806,t808,t81,t814,t815,t817,t820,t822,t823,t824,t825,t826,t827,t829,t83,t830,t831,t832,t833,t834,t835,t836,t837,t838,t84,t840,t841,t842,t843,t845,t846,t847,t848,t852,t853,t856,t86,t861,t863,t866,t868,t869,t870,t874,t875,t876,t877,t878,t880,t881,t882,t884,t885,t888,t891,t893,t894,t895,t899,t9,t90,t900,t902,t903,t905,t906,t907,t908,t909,t91,t910,t911,t912,t913,t914,t915,t916,t917,t919,t920,t921,t922,t923,t925,t926,t927,t928,t929,t930,t931,t932,t934,t935,t937,t940,t941,t942,t943,t944,t945,t946,t947,t949,t95,t950,t951,t952,t953,t954,t955,t957,t958,t961,t962,t964,t965,t968,t97,t970,t971,t972,t973,t974,t975,t976,t977,t982,t983,t984,t985,t986,t987,t988,t989,t99,t990,t991,t993,t994,t995,t998,t999});
end
function C_dq = ft_11(ct)
dq1 = ct{1};
dq2 = ct{2};
dq3 = ct{3};
dq4 = ct{4};
dq5 = ct{5};
dq6 = ct{6};
t1004 = ct{7};
t1006 = ct{8};
t1008 = ct{9};
t1013 = ct{10};
t1016 = ct{11};
t1019 = ct{12};
t1020 = ct{13};
t1023 = ct{14};
t1024 = ct{15};
t1025 = ct{16};
t1026 = ct{17};
t1028 = ct{18};
t1030 = ct{19};
t1031 = ct{20};
t1032 = ct{21};
t1034 = ct{22};
t1036 = ct{23};
t1038 = ct{24};
t1039 = ct{25};
t1040 = ct{26};
t1042 = ct{27};
t1043 = ct{28};
t1044 = ct{29};
t1045 = ct{30};
t1046 = ct{31};
t1047 = ct{32};
t1048 = ct{33};
t1049 = ct{34};
t1050 = ct{35};
t1051 = ct{36};
t1054 = ct{37};
t1055 = ct{38};
t1056 = ct{39};
t1057 = ct{40};
t1059 = ct{41};
t1061 = ct{42};
t1065 = ct{43};
t1066 = ct{44};
t1068 = ct{45};
t1069 = ct{46};
t1070 = ct{47};
t1073 = ct{48};
t1075 = ct{49};
t1076 = ct{50};
t1077 = ct{51};
t1081 = ct{52};
t1083 = ct{53};
t1084 = ct{54};
t1085 = ct{55};
t1087 = ct{56};
t1088 = ct{57};
t1089 = ct{58};
t1090 = ct{59};
t1091 = ct{60};
t1092 = ct{61};
t1093 = ct{62};
t1095 = ct{63};
t1098 = ct{64};
t1099 = ct{65};
t1101 = ct{66};
t1102 = ct{67};
t1105 = ct{68};
t1106 = ct{69};
t1107 = ct{70};
t1108 = ct{71};
t1109 = ct{72};
t111 = ct{73};
t1113 = ct{74};
t1115 = ct{75};
t1116 = ct{76};
t1119 = ct{77};
t112 = ct{78};
t1122 = ct{79};
t1125 = ct{80};
t1126 = ct{81};
t1127 = ct{82};
t1128 = ct{83};
t113 = ct{84};
t1130 = ct{85};
t1131 = ct{86};
t1133 = ct{87};
t1134 = ct{88};
t1138 = ct{89};
t1139 = ct{90};
t114 = ct{91};
t1141 = ct{92};
t1144 = ct{93};
t1146 = ct{94};
t1147 = ct{95};
t1148 = ct{96};
t115 = ct{97};
t1150 = ct{98};
t1152 = ct{99};
t1153 = ct{100};
t1155 = ct{101};
t1156 = ct{102};
t1158 = ct{103};
t1159 = ct{104};
t116 = ct{105};
t1162 = ct{106};
t1163 = ct{107};
t1165 = ct{108};
t1167 = ct{109};
t1169 = ct{110};
t1170 = ct{111};
t1171 = ct{112};
t1173 = ct{113};
t1174 = ct{114};
t1175 = ct{115};
t1177 = ct{116};
t1178 = ct{117};
t1179 = ct{118};
t1180 = ct{119};
t1181 = ct{120};
t1182 = ct{121};
t1183 = ct{122};
t1184 = ct{123};
t1185 = ct{124};
t1186 = ct{125};
t1188 = ct{126};
t1189 = ct{127};
t1190 = ct{128};
t1191 = ct{129};
t1192 = ct{130};
t1193 = ct{131};
t1194 = ct{132};
t1196 = ct{133};
t1197 = ct{134};
t1198 = ct{135};
t1199 = ct{136};
t1200 = ct{137};
t1201 = ct{138};
t1202 = ct{139};
t1203 = ct{140};
t1204 = ct{141};
t1205 = ct{142};
t1206 = ct{143};
t1207 = ct{144};
t121 = ct{145};
t1210 = ct{146};
t1211 = ct{147};
t1212 = ct{148};
t1213 = ct{149};
t1215 = ct{150};
t1219 = ct{151};
t1221 = ct{152};
t1222 = ct{153};
t1224 = ct{154};
t1225 = ct{155};
t1227 = ct{156};
t1228 = ct{157};
t1233 = ct{158};
t1235 = ct{159};
t1236 = ct{160};
t1239 = ct{161};
t1240 = ct{162};
t1244 = ct{163};
t1245 = ct{164};
t125 = ct{165};
t1250 = ct{166};
t1251 = ct{167};
t1253 = ct{168};
t1254 = ct{169};
t1256 = ct{170};
t1257 = ct{171};
t1258 = ct{172};
t1259 = ct{173};
t126 = ct{174};
t1261 = ct{175};
t1262 = ct{176};
t1263 = ct{177};
t1264 = ct{178};
t1265 = ct{179};
t1266 = ct{180};
t1267 = ct{181};
t1268 = ct{182};
t1269 = ct{183};
t1271 = ct{184};
t1272 = ct{185};
t1273 = ct{186};
t1274 = ct{187};
t1277 = ct{188};
t1278 = ct{189};
t128 = ct{190};
t1280 = ct{191};
t1282 = ct{192};
t1285 = ct{193};
t1286 = ct{194};
t1288 = ct{195};
t1289 = ct{196};
t1290 = ct{197};
t1292 = ct{198};
t1294 = ct{199};
t1295 = ct{200};
t1296 = ct{201};
t1298 = ct{202};
t1300 = ct{203};
t1301 = ct{204};
t1302 = ct{205};
t1306 = ct{206};
t1307 = ct{207};
t1308 = ct{208};
t1309 = ct{209};
t131 = ct{210};
t1311 = ct{211};
t1312 = ct{212};
t1313 = ct{213};
t1315 = ct{214};
t1316 = ct{215};
t1317 = ct{216};
t1318 = ct{217};
t1319 = ct{218};
t132 = ct{219};
t1322 = ct{220};
t1323 = ct{221};
t1324 = ct{222};
t1325 = ct{223};
t1326 = ct{224};
t1328 = ct{225};
t1329 = ct{226};
t133 = ct{227};
t1330 = ct{228};
t1331 = ct{229};
t1333 = ct{230};
t1337 = ct{231};
t1338 = ct{232};
t1340 = ct{233};
t1341 = ct{234};
t1342 = ct{235};
t1343 = ct{236};
t1344 = ct{237};
t1345 = ct{238};
t1346 = ct{239};
t1348 = ct{240};
t1351 = ct{241};
t1352 = ct{242};
t1353 = ct{243};
t1354 = ct{244};
t1355 = ct{245};
t1356 = ct{246};
t1360 = ct{247};
t1362 = ct{248};
t1365 = ct{249};
t1366 = ct{250};
t1367 = ct{251};
t1369 = ct{252};
t1370 = ct{253};
t1371 = ct{254};
t1372 = ct{255};
t1374 = ct{256};
t1375 = ct{257};
t1377 = ct{258};
t1378 = ct{259};
t1379 = ct{260};
t1380 = ct{261};
t1383 = ct{262};
t1384 = ct{263};
t1385 = ct{264};
t1386 = ct{265};
t1388 = ct{266};
t1389 = ct{267};
t139 = ct{268};
t1391 = ct{269};
t1392 = ct{270};
t1393 = ct{271};
t1394 = ct{272};
t1397 = ct{273};
t140 = ct{274};
t1401 = ct{275};
t1402 = ct{276};
t1403 = ct{277};
t1404 = ct{278};
t1406 = ct{279};
t1407 = ct{280};
t1408 = ct{281};
t1409 = ct{282};
t141 = ct{283};
t1410 = ct{284};
t1411 = ct{285};
t1413 = ct{286};
t1414 = ct{287};
t1415 = ct{288};
t1416 = ct{289};
t1417 = ct{290};
t1419 = ct{291};
t142 = ct{292};
t1423 = ct{293};
t1426 = ct{294};
t1427 = ct{295};
t1428 = ct{296};
t1429 = ct{297};
t1431 = ct{298};
t1433 = ct{299};
t1436 = ct{300};
t144 = ct{301};
t1440 = ct{302};
t1441 = ct{303};
t1442 = ct{304};
t1443 = ct{305};
t1445 = ct{306};
t1446 = ct{307};
t1447 = ct{308};
t1448 = ct{309};
t1449 = ct{310};
t1451 = ct{311};
t1452 = ct{312};
t1453 = ct{313};
t1454 = ct{314};
t1455 = ct{315};
t1456 = ct{316};
t1457 = ct{317};
t1458 = ct{318};
t1459 = ct{319};
t1460 = ct{320};
t1463 = ct{321};
t1464 = ct{322};
t1465 = ct{323};
t1470 = ct{324};
t1471 = ct{325};
t1476 = ct{326};
t1478 = ct{327};
t1479 = ct{328};
t148 = ct{329};
t1481 = ct{330};
t1482 = ct{331};
t1483 = ct{332};
t1486 = ct{333};
t1487 = ct{334};
t1488 = ct{335};
t1489 = ct{336};
t1490 = ct{337};
t1493 = ct{338};
t1494 = ct{339};
t1495 = ct{340};
t1496 = ct{341};
t1498 = ct{342};
t1499 = ct{343};
t15 = ct{344};
t150 = ct{345};
t1501 = ct{346};
t1502 = ct{347};
t1503 = ct{348};
t1505 = ct{349};
t1506 = ct{350};
t1507 = ct{351};
t1508 = ct{352};
t151 = ct{353};
t1510 = ct{354};
t1511 = ct{355};
t1512 = ct{356};
t1513 = ct{357};
t1515 = ct{358};
t1516 = ct{359};
t1517 = ct{360};
t1520 = ct{361};
t1521 = ct{362};
t1522 = ct{363};
t1523 = ct{364};
t1524 = ct{365};
t1525 = ct{366};
t1526 = ct{367};
t1527 = ct{368};
t1529 = ct{369};
t153 = ct{370};
t1530 = ct{371};
t1531 = ct{372};
t1532 = ct{373};
t1533 = ct{374};
t1534 = ct{375};
t1535 = ct{376};
t1536 = ct{377};
t1537 = ct{378};
t1538 = ct{379};
t1539 = ct{380};
t154 = ct{381};
t1540 = ct{382};
t1541 = ct{383};
t1542 = ct{384};
t1546 = ct{385};
t1548 = ct{386};
t1549 = ct{387};
t1550 = ct{388};
t1551 = ct{389};
t1553 = ct{390};
t1558 = ct{391};
t156 = ct{392};
t1560 = ct{393};
t1561 = ct{394};
t1562 = ct{395};
t1566 = ct{396};
t1567 = ct{397};
t1568 = ct{398};
t1570 = ct{399};
t1571 = ct{400};
t1572 = ct{401};
t1574 = ct{402};
t1575 = ct{403};
t1576 = ct{404};
t1577 = ct{405};
t1578 = ct{406};
t158 = ct{407};
t1580 = ct{408};
t1581 = ct{409};
t1582 = ct{410};
t1583 = ct{411};
t1584 = ct{412};
t1585 = ct{413};
t1586 = ct{414};
t1587 = ct{415};
t1589 = ct{416};
t1590 = ct{417};
t1591 = ct{418};
t1592 = ct{419};
t1593 = ct{420};
t1594 = ct{421};
t1595 = ct{422};
t1596 = ct{423};
t1597 = ct{424};
t1598 = ct{425};
t1599 = ct{426};
t16 = ct{427};
t1600 = ct{428};
t1601 = ct{429};
t1602 = ct{430};
t1605 = ct{431};
t1606 = ct{432};
t1607 = ct{433};
t1609 = ct{434};
t1610 = ct{435};
t1611 = ct{436};
t1612 = ct{437};
t1613 = ct{438};
t1614 = ct{439};
t1615 = ct{440};
t1616 = ct{441};
t1617 = ct{442};
t1618 = ct{443};
t1619 = ct{444};
t1620 = ct{445};
t1621 = ct{446};
t1622 = ct{447};
t1625 = ct{448};
t1626 = ct{449};
t1627 = ct{450};
t1628 = ct{451};
t1630 = ct{452};
t1631 = ct{453};
t1632 = ct{454};
t1633 = ct{455};
t1635 = ct{456};
t1636 = ct{457};
t1637 = ct{458};
t1638 = ct{459};
t1639 = ct{460};
t1641 = ct{461};
t1642 = ct{462};
t1643 = ct{463};
t1644 = ct{464};
t1645 = ct{465};
t1646 = ct{466};
t1647 = ct{467};
t1648 = ct{468};
t1651 = ct{469};
t1652 = ct{470};
t1653 = ct{471};
t1655 = ct{472};
t1656 = ct{473};
t1657 = ct{474};
t1658 = ct{475};
t1659 = ct{476};
t166 = ct{477};
t1660 = ct{478};
t1661 = ct{479};
t1662 = ct{480};
t1663 = ct{481};
t1666 = ct{482};
t1667 = ct{483};
t1669 = ct{484};
t1670 = ct{485};
t1671 = ct{486};
t1672 = ct{487};
t1673 = ct{488};
t1674 = ct{489};
t1675 = ct{490};
t1676 = ct{491};
t1681 = ct{492};
t1682 = ct{493};
t1683 = ct{494};
t1687 = ct{495};
t1689 = ct{496};
t1692 = ct{497};
t1696 = ct{498};
t1697 = ct{499};
t1698 = ct{500};
t1699 = ct{501};
t17 = ct{502};
t1700 = ct{503};
t1701 = ct{504};
t1702 = ct{505};
t1703 = ct{506};
t1704 = ct{507};
t1705 = ct{508};
t1706 = ct{509};
t1707 = ct{510};
t1708 = ct{511};
t1709 = ct{512};
t171 = ct{513};
t1710 = ct{514};
t1711 = ct{515};
t1712 = ct{516};
t1713 = ct{517};
t1715 = ct{518};
t1716 = ct{519};
t1718 = ct{520};
t1719 = ct{521};
t1720 = ct{522};
t1721 = ct{523};
t1722 = ct{524};
t1723 = ct{525};
t1724 = ct{526};
t1726 = ct{527};
t1728 = ct{528};
t1729 = ct{529};
t1731 = ct{530};
t1732 = ct{531};
t1733 = ct{532};
t1734 = ct{533};
t1735 = ct{534};
t1736 = ct{535};
t1737 = ct{536};
t1738 = ct{537};
t1739 = ct{538};
t1740 = ct{539};
t1741 = ct{540};
t1742 = ct{541};
t1745 = ct{542};
t1746 = ct{543};
t1747 = ct{544};
t1748 = ct{545};
t1749 = ct{546};
t1752 = ct{547};
t1753 = ct{548};
t1754 = ct{549};
t1755 = ct{550};
t1756 = ct{551};
t1757 = ct{552};
t1758 = ct{553};
t1759 = ct{554};
t1760 = ct{555};
t1761 = ct{556};
t1762 = ct{557};
t1763 = ct{558};
t1764 = ct{559};
t1765 = ct{560};
t1766 = ct{561};
t1767 = ct{562};
t1768 = ct{563};
t1769 = ct{564};
t1770 = ct{565};
t1771 = ct{566};
t1772 = ct{567};
t1774 = ct{568};
t1775 = ct{569};
t1776 = ct{570};
t1777 = ct{571};
t1779 = ct{572};
t1780 = ct{573};
t1781 = ct{574};
t1783 = ct{575};
t1784 = ct{576};
t1785 = ct{577};
t1786 = ct{578};
t1787 = ct{579};
t1788 = ct{580};
t1789 = ct{581};
t1790 = ct{582};
t1791 = ct{583};
t1792 = ct{584};
t1793 = ct{585};
t1794 = ct{586};
t1795 = ct{587};
t1797 = ct{588};
t1798 = ct{589};
t1799 = ct{590};
t18 = ct{591};
t1800 = ct{592};
t1801 = ct{593};
t1804 = ct{594};
t1805 = ct{595};
t1806 = ct{596};
t1807 = ct{597};
t1808 = ct{598};
t1809 = ct{599};
t1810 = ct{600};
t1811 = ct{601};
t1812 = ct{602};
t1813 = ct{603};
t1814 = ct{604};
t1815 = ct{605};
t1816 = ct{606};
t1817 = ct{607};
t1820 = ct{608};
t1821 = ct{609};
t1822 = ct{610};
t1823 = ct{611};
t1824 = ct{612};
t1827 = ct{613};
t1828 = ct{614};
t1829 = ct{615};
t183 = ct{616};
t1830 = ct{617};
t1831 = ct{618};
t1832 = ct{619};
t1833 = ct{620};
t1834 = ct{621};
t1835 = ct{622};
t1836 = ct{623};
t1837 = ct{624};
t1838 = ct{625};
t1839 = ct{626};
t1844 = ct{627};
t1847 = ct{628};
t1848 = ct{629};
t1849 = ct{630};
t185 = ct{631};
t1850 = ct{632};
t1851 = ct{633};
t1853 = ct{634};
t1855 = ct{635};
t1856 = ct{636};
t1857 = ct{637};
t1858 = ct{638};
t1859 = ct{639};
t1860 = ct{640};
t1861 = ct{641};
t1863 = ct{642};
t1864 = ct{643};
t1865 = ct{644};
t1866 = ct{645};
t1867 = ct{646};
t1868 = ct{647};
t1870 = ct{648};
t1871 = ct{649};
t1873 = ct{650};
t1877 = ct{651};
t1878 = ct{652};
t1879 = ct{653};
t1881 = ct{654};
t1882 = ct{655};
t1884 = ct{656};
t1885 = ct{657};
t1886 = ct{658};
t1887 = ct{659};
t1889 = ct{660};
t1891 = ct{661};
t1892 = ct{662};
t1893 = ct{663};
t1896 = ct{664};
t1899 = ct{665};
t19 = ct{666};
t190 = ct{667};
t1900 = ct{668};
t1901 = ct{669};
t1902 = ct{670};
t1903 = ct{671};
t1905 = ct{672};
t1906 = ct{673};
t1907 = ct{674};
t1908 = ct{675};
t1909 = ct{676};
t191 = ct{677};
t1910 = ct{678};
t1911 = ct{679};
t1912 = ct{680};
t1913 = ct{681};
t1914 = ct{682};
t1915 = ct{683};
t1916 = ct{684};
t1917 = ct{685};
t1918 = ct{686};
t1919 = ct{687};
t1920 = ct{688};
t1921 = ct{689};
t1922 = ct{690};
t1925 = ct{691};
t1926 = ct{692};
t1927 = ct{693};
t1928 = ct{694};
t1929 = ct{695};
t1930 = ct{696};
t1935 = ct{697};
t1936 = ct{698};
t1937 = ct{699};
t1938 = ct{700};
t1939 = ct{701};
t1940 = ct{702};
t1941 = ct{703};
t1942 = ct{704};
t1943 = ct{705};
t1944 = ct{706};
t1946 = ct{707};
t1947 = ct{708};
t1950 = ct{709};
t1951 = ct{710};
t1952 = ct{711};
t1953 = ct{712};
t1954 = ct{713};
t1955 = ct{714};
t196 = ct{715};
t1961 = ct{716};
t1966 = ct{717};
t1967 = ct{718};
t1968 = ct{719};
t1969 = ct{720};
t197 = ct{721};
t1970 = ct{722};
t1971 = ct{723};
t1974 = ct{724};
t1975 = ct{725};
t1976 = ct{726};
t1977 = ct{727};
t1978 = ct{728};
t1979 = ct{729};
t1980 = ct{730};
t1981 = ct{731};
t1983 = ct{732};
t1984 = ct{733};
t1985 = ct{734};
t1986 = ct{735};
t1987 = ct{736};
t1988 = ct{737};
t1989 = ct{738};
t199 = ct{739};
t1990 = ct{740};
t1991 = ct{741};
t1992 = ct{742};
t1993 = ct{743};
t1994 = ct{744};
t1995 = ct{745};
t1996 = ct{746};
t1997 = ct{747};
t1998 = ct{748};
t1999 = ct{749};
t2 = ct{750};
t20 = ct{751};
t200 = ct{752};
t2000 = ct{753};
t2001 = ct{754};
t2002 = ct{755};
t2003 = ct{756};
t2004 = ct{757};
t2005 = ct{758};
t2006 = ct{759};
t2008 = ct{760};
t201 = ct{761};
t2010 = ct{762};
t2011 = ct{763};
t2014 = ct{764};
t2015 = ct{765};
t2016 = ct{766};
t2017 = ct{767};
t2018 = ct{768};
t2019 = ct{769};
t202 = ct{770};
t2020 = ct{771};
t2023 = ct{772};
t2024 = ct{773};
t2026 = ct{774};
t2027 = ct{775};
t2028 = ct{776};
t2029 = ct{777};
t203 = ct{778};
t2033 = ct{779};
t2034 = ct{780};
t2035 = ct{781};
t2036 = ct{782};
t2037 = ct{783};
t2038 = ct{784};
t2039 = ct{785};
t204 = ct{786};
t2040 = ct{787};
t2042 = ct{788};
t2043 = ct{789};
t2045 = ct{790};
t2047 = ct{791};
t205 = ct{792};
t2050 = ct{793};
t2051 = ct{794};
t2052 = ct{795};
t2053 = ct{796};
t2054 = ct{797};
t2056 = ct{798};
t2057 = ct{799};
t2058 = ct{800};
t2059 = ct{801};
t206 = ct{802};
t2060 = ct{803};
t2061 = ct{804};
t2062 = ct{805};
t2065 = ct{806};
t2066 = ct{807};
t2067 = ct{808};
t2068 = ct{809};
t2069 = ct{810};
t207 = ct{811};
t2070 = ct{812};
t2071 = ct{813};
t2072 = ct{814};
t2073 = ct{815};
t2074 = ct{816};
t2075 = ct{817};
t2076 = ct{818};
t2077 = ct{819};
t2078 = ct{820};
t2079 = ct{821};
t2081 = ct{822};
t2082 = ct{823};
t2083 = ct{824};
t2084 = ct{825};
t2085 = ct{826};
t2086 = ct{827};
t2087 = ct{828};
t2088 = ct{829};
t2089 = ct{830};
t209 = ct{831};
t2090 = ct{832};
t2091 = ct{833};
t2092 = ct{834};
t2093 = ct{835};
t2094 = ct{836};
t2095 = ct{837};
t2096 = ct{838};
t2097 = ct{839};
t2098 = ct{840};
t2099 = ct{841};
t21 = ct{842};
t210 = ct{843};
t2100 = ct{844};
t2101 = ct{845};
t2104 = ct{846};
t2105 = ct{847};
t2106 = ct{848};
t2107 = ct{849};
t2108 = ct{850};
t2109 = ct{851};
t211 = ct{852};
t2110 = ct{853};
t2111 = ct{854};
t2113 = ct{855};
t2114 = ct{856};
t2115 = ct{857};
t2116 = ct{858};
t2117 = ct{859};
t2118 = ct{860};
t2119 = ct{861};
t2121 = ct{862};
t2123 = ct{863};
t2125 = ct{864};
t2127 = ct{865};
t2128 = ct{866};
t2129 = ct{867};
t213 = ct{868};
t2130 = ct{869};
t2131 = ct{870};
t2132 = ct{871};
t2133 = ct{872};
t2134 = ct{873};
t2135 = ct{874};
t2136 = ct{875};
t2137 = ct{876};
t2138 = ct{877};
t214 = ct{878};
t2142 = ct{879};
t2143 = ct{880};
t2144 = ct{881};
t2145 = ct{882};
t2146 = ct{883};
t2148 = ct{884};
t2149 = ct{885};
t2150 = ct{886};
t2151 = ct{887};
t2152 = ct{888};
t2154 = ct{889};
t2155 = ct{890};
t2156 = ct{891};
t2157 = ct{892};
t2158 = ct{893};
t2159 = ct{894};
t2164 = ct{895};
t2165 = ct{896};
t2166 = ct{897};
t2169 = ct{898};
t217 = ct{899};
t2170 = ct{900};
t2171 = ct{901};
t2172 = ct{902};
t2174 = ct{903};
t2175 = ct{904};
t2176 = ct{905};
t2177 = ct{906};
t2178 = ct{907};
t2180 = ct{908};
t2181 = ct{909};
t2182 = ct{910};
t2184 = ct{911};
t2185 = ct{912};
t2186 = ct{913};
t2187 = ct{914};
t2189 = ct{915};
t2190 = ct{916};
t2191 = ct{917};
t2192 = ct{918};
t2193 = ct{919};
t2194 = ct{920};
t2196 = ct{921};
t2197 = ct{922};
t2198 = ct{923};
t2199 = ct{924};
t22 = ct{925};
t2200 = ct{926};
t2201 = ct{927};
t2202 = ct{928};
t2203 = ct{929};
t2204 = ct{930};
t2208 = ct{931};
t2209 = ct{932};
t2211 = ct{933};
t2212 = ct{934};
t2213 = ct{935};
t2214 = ct{936};
t2215 = ct{937};
t2216 = ct{938};
t2217 = ct{939};
t2218 = ct{940};
t2219 = ct{941};
t2220 = ct{942};
t2221 = ct{943};
t2223 = ct{944};
t2224 = ct{945};
t2225 = ct{946};
t2227 = ct{947};
t2228 = ct{948};
t2229 = ct{949};
t2230 = ct{950};
t2231 = ct{951};
t2232 = ct{952};
t2233 = ct{953};
t2234 = ct{954};
t2236 = ct{955};
t2237 = ct{956};
t2238 = ct{957};
t2239 = ct{958};
t224 = ct{959};
t2240 = ct{960};
t2241 = ct{961};
t2242 = ct{962};
t2243 = ct{963};
t2246 = ct{964};
t2247 = ct{965};
t2248 = ct{966};
t2249 = ct{967};
t225 = ct{968};
t2251 = ct{969};
t2253 = ct{970};
t2254 = ct{971};
t2256 = ct{972};
t2257 = ct{973};
t2258 = ct{974};
t2263 = ct{975};
t2264 = ct{976};
t2265 = ct{977};
t2266 = ct{978};
t2267 = ct{979};
t2268 = ct{980};
t2269 = ct{981};
t227 = ct{982};
t2270 = ct{983};
t2271 = ct{984};
t2272 = ct{985};
t2273 = ct{986};
t2274 = ct{987};
t2276 = ct{988};
t2277 = ct{989};
t2278 = ct{990};
t2279 = ct{991};
t228 = ct{992};
t2280 = ct{993};
t2281 = ct{994};
t2282 = ct{995};
t2283 = ct{996};
t2284 = ct{997};
t2285 = ct{998};
t2286 = ct{999};
t2288 = ct{1000};
t2289 = ct{1001};
t2290 = ct{1002};
t2291 = ct{1003};
t2295 = ct{1004};
t2296 = ct{1005};
t2297 = ct{1006};
t2298 = ct{1007};
t2299 = ct{1008};
t23 = ct{1009};
t230 = ct{1010};
t2300 = ct{1011};
t2302 = ct{1012};
t2303 = ct{1013};
t2304 = ct{1014};
t2305 = ct{1015};
t2306 = ct{1016};
t2307 = ct{1017};
t2308 = ct{1018};
t231 = ct{1019};
t2310 = ct{1020};
t2311 = ct{1021};
t2312 = ct{1022};
t2313 = ct{1023};
t2314 = ct{1024};
t2315 = ct{1025};
t2316 = ct{1026};
t2317 = ct{1027};
t2318 = ct{1028};
t2319 = ct{1029};
t2320 = ct{1030};
t2321 = ct{1031};
t2322 = ct{1032};
t2323 = ct{1033};
t2324 = ct{1034};
t2326 = ct{1035};
t2327 = ct{1036};
t2328 = ct{1037};
t233 = ct{1038};
t2330 = ct{1039};
t2331 = ct{1040};
t2332 = ct{1041};
t2333 = ct{1042};
t2334 = ct{1043};
t2336 = ct{1044};
t2337 = ct{1045};
t2338 = ct{1046};
t2339 = ct{1047};
t234 = ct{1048};
t2340 = ct{1049};
t2341 = ct{1050};
t2342 = ct{1051};
t2344 = ct{1052};
t2345 = ct{1053};
t2346 = ct{1054};
t2347 = ct{1055};
t2348 = ct{1056};
t235 = ct{1057};
t2350 = ct{1058};
t2354 = ct{1059};
t2355 = ct{1060};
t2357 = ct{1061};
t2358 = ct{1062};
t2359 = ct{1063};
t236 = ct{1064};
t2361 = ct{1065};
t2362 = ct{1066};
t2363 = ct{1067};
t2364 = ct{1068};
t2365 = ct{1069};
t2366 = ct{1070};
t2367 = ct{1071};
t2369 = ct{1072};
t2370 = ct{1073};
t2371 = ct{1074};
t2372 = ct{1075};
t2373 = ct{1076};
t2374 = ct{1077};
t2375 = ct{1078};
t2376 = ct{1079};
t2377 = ct{1080};
t2378 = ct{1081};
t2379 = ct{1082};
t2382 = ct{1083};
t2383 = ct{1084};
t2384 = ct{1085};
t2385 = ct{1086};
t2386 = ct{1087};
t2387 = ct{1088};
t2388 = ct{1089};
t2389 = ct{1090};
t2390 = ct{1091};
t2391 = ct{1092};
t2392 = ct{1093};
t2393 = ct{1094};
t2394 = ct{1095};
t2395 = ct{1096};
t2396 = ct{1097};
t2397 = ct{1098};
t2398 = ct{1099};
t24 = ct{1100};
t240 = ct{1101};
t2400 = ct{1102};
t2401 = ct{1103};
t2402 = ct{1104};
t2403 = ct{1105};
t2404 = ct{1106};
t2405 = ct{1107};
t2406 = ct{1108};
t2407 = ct{1109};
t2408 = ct{1110};
t2410 = ct{1111};
t2416 = ct{1112};
t2417 = ct{1113};
t2420 = ct{1114};
t2421 = ct{1115};
t2422 = ct{1116};
t2424 = ct{1117};
t2425 = ct{1118};
t2426 = ct{1119};
t2427 = ct{1120};
t2428 = ct{1121};
t2429 = ct{1122};
t243 = ct{1123};
t2430 = ct{1124};
t2431 = ct{1125};
t2434 = ct{1126};
t2435 = ct{1127};
t2437 = ct{1128};
t2438 = ct{1129};
t2439 = ct{1130};
t244 = ct{1131};
t2440 = ct{1132};
t2441 = ct{1133};
t2443 = ct{1134};
t2444 = ct{1135};
t2446 = ct{1136};
t2448 = ct{1137};
t2449 = ct{1138};
t2452 = ct{1139};
t2453 = ct{1140};
t2454 = ct{1141};
t2455 = ct{1142};
t2456 = ct{1143};
t2457 = ct{1144};
t2458 = ct{1145};
t2460 = ct{1146};
t2463 = ct{1147};
t2465 = ct{1148};
t2466 = ct{1149};
t2467 = ct{1150};
t2470 = ct{1151};
t2473 = ct{1152};
t2474 = ct{1153};
t2477 = ct{1154};
t2478 = ct{1155};
t2479 = ct{1156};
t2481 = ct{1157};
t2483 = ct{1158};
t2484 = ct{1159};
t2485 = ct{1160};
t2486 = ct{1161};
t2487 = ct{1162};
t2489 = ct{1163};
t249 = ct{1164};
t2490 = ct{1165};
t2494 = ct{1166};
t2495 = ct{1167};
t2497 = ct{1168};
t2500 = ct{1169};
t2502 = ct{1170};
t2503 = ct{1171};
t2505 = ct{1172};
t2507 = ct{1173};
t2508 = ct{1174};
t2510 = ct{1175};
t2511 = ct{1176};
t2512 = ct{1177};
t2513 = ct{1178};
t2517 = ct{1179};
t2518 = ct{1180};
t2519 = ct{1181};
t2520 = ct{1182};
t2521 = ct{1183};
t2522 = ct{1184};
t2523 = ct{1185};
t2524 = ct{1186};
t2525 = ct{1187};
t2526 = ct{1188};
t2527 = ct{1189};
t2530 = ct{1190};
t2531 = ct{1191};
t2533 = ct{1192};
t2534 = ct{1193};
t2535 = ct{1194};
t2536 = ct{1195};
t2537 = ct{1196};
t2539 = ct{1197};
t2540 = ct{1198};
t2541 = ct{1199};
t2542 = ct{1200};
t2543 = ct{1201};
t2544 = ct{1202};
t2545 = ct{1203};
t2546 = ct{1204};
t2547 = ct{1205};
t2548 = ct{1206};
t2549 = ct{1207};
t2552 = ct{1208};
t2553 = ct{1209};
t2554 = ct{1210};
t2555 = ct{1211};
t2556 = ct{1212};
t2560 = ct{1213};
t2562 = ct{1214};
t2563 = ct{1215};
t2564 = ct{1216};
t2565 = ct{1217};
t2566 = ct{1218};
t2567 = ct{1219};
t2568 = ct{1220};
t2569 = ct{1221};
t257 = ct{1222};
t2570 = ct{1223};
t2571 = ct{1224};
t2574 = ct{1225};
t2575 = ct{1226};
t2576 = ct{1227};
t2577 = ct{1228};
t2578 = ct{1229};
t2579 = ct{1230};
t258 = ct{1231};
t2581 = ct{1232};
t2582 = ct{1233};
t2585 = ct{1234};
t2586 = ct{1235};
t2587 = ct{1236};
t2588 = ct{1237};
t2589 = ct{1238};
t2590 = ct{1239};
t2594 = ct{1240};
t2595 = ct{1241};
t2597 = ct{1242};
t2598 = ct{1243};
t2599 = ct{1244};
t2602 = ct{1245};
t2603 = ct{1246};
t2604 = ct{1247};
t2606 = ct{1248};
t2607 = ct{1249};
t2608 = ct{1250};
t2611 = ct{1251};
t2612 = ct{1252};
t2613 = ct{1253};
t2614 = ct{1254};
t2615 = ct{1255};
t2616 = ct{1256};
t2617 = ct{1257};
t2620 = ct{1258};
t2622 = ct{1259};
t2623 = ct{1260};
t2624 = ct{1261};
t2625 = ct{1262};
t2626 = ct{1263};
t2627 = ct{1264};
t2628 = ct{1265};
t2629 = ct{1266};
t263 = ct{1267};
t2630 = ct{1268};
t2631 = ct{1269};
t2633 = ct{1270};
t2634 = ct{1271};
t2636 = ct{1272};
t2639 = ct{1273};
t2640 = ct{1274};
t2641 = ct{1275};
t2644 = ct{1276};
t2647 = ct{1277};
t2648 = ct{1278};
t2649 = ct{1279};
t2650 = ct{1280};
t2651 = ct{1281};
t2654 = ct{1282};
t2655 = ct{1283};
t2656 = ct{1284};
t2657 = ct{1285};
t2659 = ct{1286};
t266 = ct{1287};
t2660 = ct{1288};
t2661 = ct{1289};
t2662 = ct{1290};
t2663 = ct{1291};
t2664 = ct{1292};
t2665 = ct{1293};
t2666 = ct{1294};
t2668 = ct{1295};
t2669 = ct{1296};
t2670 = ct{1297};
t2671 = ct{1298};
t2673 = ct{1299};
t2675 = ct{1300};
t2676 = ct{1301};
t2677 = ct{1302};
t2678 = ct{1303};
t2679 = ct{1304};
t2680 = ct{1305};
t2681 = ct{1306};
t2682 = ct{1307};
t2684 = ct{1308};
t2685 = ct{1309};
t2686 = ct{1310};
t2688 = ct{1311};
t2689 = ct{1312};
t2691 = ct{1313};
t2692 = ct{1314};
t2693 = ct{1315};
t2694 = ct{1316};
t2695 = ct{1317};
t2696 = ct{1318};
t2697 = ct{1319};
t2698 = ct{1320};
t2699 = ct{1321};
t270 = ct{1322};
t2700 = ct{1323};
t2701 = ct{1324};
t2705 = ct{1325};
t2706 = ct{1326};
t2707 = ct{1327};
t2708 = ct{1328};
t2711 = ct{1329};
t2712 = ct{1330};
t2713 = ct{1331};
t2714 = ct{1332};
t2715 = ct{1333};
t2718 = ct{1334};
t2719 = ct{1335};
t2720 = ct{1336};
t2721 = ct{1337};
t2722 = ct{1338};
t2723 = ct{1339};
t2724 = ct{1340};
t2725 = ct{1341};
t2726 = ct{1342};
t2728 = ct{1343};
t2729 = ct{1344};
t273 = ct{1345};
t2730 = ct{1346};
t2731 = ct{1347};
t2732 = ct{1348};
t2735 = ct{1349};
t2736 = ct{1350};
t2737 = ct{1351};
t2738 = ct{1352};
t274 = ct{1353};
t2740 = ct{1354};
t2741 = ct{1355};
t2742 = ct{1356};
t2743 = ct{1357};
t2744 = ct{1358};
t2746 = ct{1359};
t2747 = ct{1360};
t2748 = ct{1361};
t2749 = ct{1362};
t275 = ct{1363};
t2750 = ct{1364};
t2752 = ct{1365};
t2753 = ct{1366};
t2754 = ct{1367};
t2755 = ct{1368};
t2756 = ct{1369};
t2757 = ct{1370};
t2758 = ct{1371};
t2759 = ct{1372};
t276 = ct{1373};
t2760 = ct{1374};
t2761 = ct{1375};
t2762 = ct{1376};
t2763 = ct{1377};
t2764 = ct{1378};
t2765 = ct{1379};
t2766 = ct{1380};
t2767 = ct{1381};
t2769 = ct{1382};
t277 = ct{1383};
t2770 = ct{1384};
t2771 = ct{1385};
t2772 = ct{1386};
t2774 = ct{1387};
t2775 = ct{1388};
t2777 = ct{1389};
t2778 = ct{1390};
t278 = ct{1391};
t2780 = ct{1392};
t2783 = ct{1393};
t2784 = ct{1394};
t2785 = ct{1395};
t2791 = ct{1396};
t2792 = ct{1397};
t2793 = ct{1398};
t2795 = ct{1399};
t2796 = ct{1400};
t2797 = ct{1401};
t2798 = ct{1402};
t2799 = ct{1403};
t280 = ct{1404};
t2800 = ct{1405};
t2801 = ct{1406};
t2802 = ct{1407};
t2803 = ct{1408};
t2805 = ct{1409};
t2806 = ct{1410};
t2807 = ct{1411};
t2809 = ct{1412};
t2812 = ct{1413};
t2814 = ct{1414};
t2815 = ct{1415};
t2816 = ct{1416};
t2817 = ct{1417};
t2818 = ct{1418};
t2819 = ct{1419};
t2820 = ct{1420};
t2822 = ct{1421};
t2823 = ct{1422};
t2824 = ct{1423};
t2825 = ct{1424};
t2826 = ct{1425};
t2827 = ct{1426};
t2828 = ct{1427};
t2829 = ct{1428};
t2830 = ct{1429};
t2831 = ct{1430};
t2832 = ct{1431};
t2833 = ct{1432};
t2834 = ct{1433};
t2835 = ct{1434};
t2836 = ct{1435};
t2839 = ct{1436};
t284 = ct{1437};
t2842 = ct{1438};
t2844 = ct{1439};
t2845 = ct{1440};
t2846 = ct{1441};
t2850 = ct{1442};
t2851 = ct{1443};
t2852 = ct{1444};
t2854 = ct{1445};
t2857 = ct{1446};
t2861 = ct{1447};
t2863 = ct{1448};
t2864 = ct{1449};
t2867 = ct{1450};
t2868 = ct{1451};
t2869 = ct{1452};
t287 = ct{1453};
t2872 = ct{1454};
t2877 = ct{1455};
t2878 = ct{1456};
t2880 = ct{1457};
t2881 = ct{1458};
t2882 = ct{1459};
t2883 = ct{1460};
t2884 = ct{1461};
t2885 = ct{1462};
t2886 = ct{1463};
t2887 = ct{1464};
t2888 = ct{1465};
t2889 = ct{1466};
t2892 = ct{1467};
t2893 = ct{1468};
t2894 = ct{1469};
t2895 = ct{1470};
t2896 = ct{1471};
t2897 = ct{1472};
t29 = ct{1473};
t290 = ct{1474};
t2900 = ct{1475};
t2903 = ct{1476};
t2904 = ct{1477};
t2905 = ct{1478};
t2906 = ct{1479};
t2907 = ct{1480};
t2908 = ct{1481};
t2909 = ct{1482};
t291 = ct{1483};
t2910 = ct{1484};
t2911 = ct{1485};
t2912 = ct{1486};
t2913 = ct{1487};
t2914 = ct{1488};
t2915 = ct{1489};
t2916 = ct{1490};
t2917 = ct{1491};
t2918 = ct{1492};
t2919 = ct{1493};
t292 = ct{1494};
t2920 = ct{1495};
t2921 = ct{1496};
t2922 = ct{1497};
t2923 = ct{1498};
t2925 = ct{1499};
t2928 = ct{1500};
t2929 = ct{1501};
t2930 = ct{1502};
t2931 = ct{1503};
t2932 = ct{1504};
t2933 = ct{1505};
t2937 = ct{1506};
t294 = ct{1507};
t2940 = ct{1508};
t2941 = ct{1509};
t2942 = ct{1510};
t2944 = ct{1511};
t2945 = ct{1512};
t2946 = ct{1513};
t2947 = ct{1514};
t2949 = ct{1515};
t2950 = ct{1516};
t2951 = ct{1517};
t2952 = ct{1518};
t2956 = ct{1519};
t2958 = ct{1520};
t2959 = ct{1521};
t2962 = ct{1522};
t2965 = ct{1523};
t2966 = ct{1524};
t2967 = ct{1525};
t2968 = ct{1526};
t2969 = ct{1527};
t297 = ct{1528};
t2970 = ct{1529};
t2971 = ct{1530};
t2972 = ct{1531};
t2973 = ct{1532};
t2975 = ct{1533};
t2977 = ct{1534};
t2978 = ct{1535};
t2980 = ct{1536};
t2983 = ct{1537};
t2984 = ct{1538};
t2985 = ct{1539};
t2986 = ct{1540};
t2987 = ct{1541};
t2988 = ct{1542};
t2989 = ct{1543};
t299 = ct{1544};
t2991 = ct{1545};
t2992 = ct{1546};
t2993 = ct{1547};
t2994 = ct{1548};
t2995 = ct{1549};
t2996 = ct{1550};
t2997 = ct{1551};
t2998 = ct{1552};
t2999 = ct{1553};
t3 = ct{1554};
t30 = ct{1555};
t300 = ct{1556};
t3000 = ct{1557};
t3001 = ct{1558};
t3002 = ct{1559};
t3003 = ct{1560};
t3005 = ct{1561};
t3007 = ct{1562};
t3008 = ct{1563};
t3010 = ct{1564};
t3011 = ct{1565};
t3013 = ct{1566};
t3014 = ct{1567};
t3015 = ct{1568};
t3018 = ct{1569};
t3019 = ct{1570};
t302 = ct{1571};
t3020 = ct{1572};
t3021 = ct{1573};
t3022 = ct{1574};
t3024 = ct{1575};
t3025 = ct{1576};
t3027 = ct{1577};
t3029 = ct{1578};
t303 = ct{1579};
t3030 = ct{1580};
t3031 = ct{1581};
t3032 = ct{1582};
t3033 = ct{1583};
t3034 = ct{1584};
t3035 = ct{1585};
t3036 = ct{1586};
t3037 = ct{1587};
t3038 = ct{1588};
t304 = ct{1589};
t3041 = ct{1590};
t3043 = ct{1591};
t3044 = ct{1592};
t3046 = ct{1593};
t3047 = ct{1594};
t3048 = ct{1595};
t3049 = ct{1596};
t305 = ct{1597};
t3050 = ct{1598};
t3051 = ct{1599};
t3052 = ct{1600};
t3053 = ct{1601};
t3054 = ct{1602};
t3055 = ct{1603};
t3056 = ct{1604};
t3057 = ct{1605};
t3059 = ct{1606};
t306 = ct{1607};
t3060 = ct{1608};
t3061 = ct{1609};
t3062 = ct{1610};
t3064 = ct{1611};
t3065 = ct{1612};
t3066 = ct{1613};
t3067 = ct{1614};
t3068 = ct{1615};
t3069 = ct{1616};
t3070 = ct{1617};
t3071 = ct{1618};
t3072 = ct{1619};
t3073 = ct{1620};
t3074 = ct{1621};
t3076 = ct{1622};
t3077 = ct{1623};
t3079 = ct{1624};
t3080 = ct{1625};
t3081 = ct{1626};
t3082 = ct{1627};
t3083 = ct{1628};
t3084 = ct{1629};
t3085 = ct{1630};
t3086 = ct{1631};
t3088 = ct{1632};
t3089 = ct{1633};
t309 = ct{1634};
t3090 = ct{1635};
t3092 = ct{1636};
t3094 = ct{1637};
t3095 = ct{1638};
t3096 = ct{1639};
t3097 = ct{1640};
t3098 = ct{1641};
t3099 = ct{1642};
t310 = ct{1643};
t3100 = ct{1644};
t3103 = ct{1645};
t3104 = ct{1646};
t3105 = ct{1647};
t3106 = ct{1648};
t3108 = ct{1649};
t3109 = ct{1650};
t311 = ct{1651};
t3110 = ct{1652};
t3112 = ct{1653};
t3113 = ct{1654};
t3114 = ct{1655};
t3117 = ct{1656};
t3118 = ct{1657};
t3119 = ct{1658};
t3120 = ct{1659};
t3121 = ct{1660};
t3122 = ct{1661};
t3123 = ct{1662};
t3124 = ct{1663};
t3125 = ct{1664};
t3126 = ct{1665};
t3127 = ct{1666};
t3128 = ct{1667};
t3129 = ct{1668};
t313 = ct{1669};
t3130 = ct{1670};
t3131 = ct{1671};
t3132 = ct{1672};
t3133 = ct{1673};
t3134 = ct{1674};
t3136 = ct{1675};
t3139 = ct{1676};
t314 = ct{1677};
t3140 = ct{1678};
t3142 = ct{1679};
t3143 = ct{1680};
t3146 = ct{1681};
t3148 = ct{1682};
t3149 = ct{1683};
t315 = ct{1684};
t3150 = ct{1685};
t3152 = ct{1686};
t3153 = ct{1687};
t3154 = ct{1688};
t3156 = ct{1689};
t3157 = ct{1690};
t3158 = ct{1691};
t3159 = ct{1692};
t316 = ct{1693};
t3160 = ct{1694};
t3161 = ct{1695};
t3163 = ct{1696};
t3164 = ct{1697};
t3166 = ct{1698};
t3167 = ct{1699};
t3168 = ct{1700};
t3169 = ct{1701};
t3170 = ct{1702};
t3171 = ct{1703};
t3172 = ct{1704};
t3174 = ct{1705};
t3175 = ct{1706};
t3176 = ct{1707};
t3178 = ct{1708};
t3179 = ct{1709};
t318 = ct{1710};
t3180 = ct{1711};
t3182 = ct{1712};
t3183 = ct{1713};
t3184 = ct{1714};
t3185 = ct{1715};
t3186 = ct{1716};
t3187 = ct{1717};
t3188 = ct{1718};
t3189 = ct{1719};
t319 = ct{1720};
t3190 = ct{1721};
t3191 = ct{1722};
t3192 = ct{1723};
t3193 = ct{1724};
t3194 = ct{1725};
t3195 = ct{1726};
t3196 = ct{1727};
t3198 = ct{1728};
t3199 = ct{1729};
t320 = ct{1730};
t3200 = ct{1731};
t3207 = ct{1732};
t3208 = ct{1733};
t3209 = ct{1734};
t3210 = ct{1735};
t3213 = ct{1736};
t3217 = ct{1737};
t3219 = ct{1738};
t322 = ct{1739};
t3220 = ct{1740};
t3221 = ct{1741};
t3222 = ct{1742};
t3223 = ct{1743};
t3224 = ct{1744};
t3228 = ct{1745};
t3229 = ct{1746};
t3230 = ct{1747};
t3232 = ct{1748};
t3234 = ct{1749};
t3236 = ct{1750};
t3237 = ct{1751};
t3238 = ct{1752};
t3239 = ct{1753};
t324 = ct{1754};
t3240 = ct{1755};
t3245 = ct{1756};
t3246 = ct{1757};
t3247 = ct{1758};
t3248 = ct{1759};
t325 = ct{1760};
t3250 = ct{1761};
t3251 = ct{1762};
t3252 = ct{1763};
t3254 = ct{1764};
t3265 = ct{1765};
t3266 = ct{1766};
t3267 = ct{1767};
t3268 = ct{1768};
t3269 = ct{1769};
t3270 = ct{1770};
t3271 = ct{1771};
t3272 = ct{1772};
t3273 = ct{1773};
t3274 = ct{1774};
t3275 = ct{1775};
t3277 = ct{1776};
t3278 = ct{1777};
t3279 = ct{1778};
t328 = ct{1779};
t3280 = ct{1780};
t3282 = ct{1781};
t3283 = ct{1782};
t3284 = ct{1783};
t3285 = ct{1784};
t3286 = ct{1785};
t3287 = ct{1786};
t3288 = ct{1787};
t3289 = ct{1788};
t3290 = ct{1789};
t3291 = ct{1790};
t3292 = ct{1791};
t3293 = ct{1792};
t3295 = ct{1793};
t3296 = ct{1794};
t3297 = ct{1795};
t3298 = ct{1796};
t3299 = ct{1797};
t3301 = ct{1798};
t3302 = ct{1799};
t3303 = ct{1800};
t3306 = ct{1801};
t3307 = ct{1802};
t3308 = ct{1803};
t3309 = ct{1804};
t3310 = ct{1805};
t3312 = ct{1806};
t3313 = ct{1807};
t3314 = ct{1808};
t3317 = ct{1809};
t3318 = ct{1810};
t3320 = ct{1811};
t3321 = ct{1812};
t3322 = ct{1813};
t3323 = ct{1814};
t3324 = ct{1815};
t3325 = ct{1816};
t3326 = ct{1817};
t3327 = ct{1818};
t3328 = ct{1819};
t3329 = ct{1820};
t333 = ct{1821};
t3331 = ct{1822};
t3332 = ct{1823};
t3333 = ct{1824};
t3334 = ct{1825};
t3335 = ct{1826};
t3336 = ct{1827};
t3337 = ct{1828};
t3338 = ct{1829};
t3339 = ct{1830};
t3340 = ct{1831};
t3341 = ct{1832};
t3342 = ct{1833};
t3343 = ct{1834};
t3346 = ct{1835};
t3347 = ct{1836};
t3349 = ct{1837};
t3350 = ct{1838};
t3351 = ct{1839};
t3352 = ct{1840};
t3353 = ct{1841};
t3354 = ct{1842};
t3356 = ct{1843};
t3357 = ct{1844};
t3358 = ct{1845};
t3359 = ct{1846};
t336 = ct{1847};
t3360 = ct{1848};
t3362 = ct{1849};
t3363 = ct{1850};
t3364 = ct{1851};
t3365 = ct{1852};
t3366 = ct{1853};
t3367 = ct{1854};
t3368 = ct{1855};
t3369 = ct{1856};
t337 = ct{1857};
t3371 = ct{1858};
t3372 = ct{1859};
t3373 = ct{1860};
t3374 = ct{1861};
t3375 = ct{1862};
t3376 = ct{1863};
t3377 = ct{1864};
t3378 = ct{1865};
t3380 = ct{1866};
t3381 = ct{1867};
t3382 = ct{1868};
t3383 = ct{1869};
t3384 = ct{1870};
t3386 = ct{1871};
t3387 = ct{1872};
t3388 = ct{1873};
t3390 = ct{1874};
t3391 = ct{1875};
t3392 = ct{1876};
t3393 = ct{1877};
t3394 = ct{1878};
t3395 = ct{1879};
t3396 = ct{1880};
t3397 = ct{1881};
t3398 = ct{1882};
t3399 = ct{1883};
t34 = ct{1884};
t340 = ct{1885};
t3400 = ct{1886};
t3402 = ct{1887};
t3403 = ct{1888};
t3404 = ct{1889};
t3405 = ct{1890};
t3407 = ct{1891};
t3408 = ct{1892};
t3409 = ct{1893};
t3410 = ct{1894};
t3411 = ct{1895};
t3412 = ct{1896};
t3413 = ct{1897};
t3416 = ct{1898};
t3417 = ct{1899};
t3418 = ct{1900};
t3420 = ct{1901};
t3421 = ct{1902};
t3422 = ct{1903};
t3423 = ct{1904};
t3424 = ct{1905};
t3425 = ct{1906};
t3426 = ct{1907};
t3427 = ct{1908};
t3429 = ct{1909};
t3430 = ct{1910};
t3431 = ct{1911};
t3432 = ct{1912};
t3433 = ct{1913};
t3434 = ct{1914};
t3435 = ct{1915};
t3436 = ct{1916};
t3437 = ct{1917};
t3439 = ct{1918};
t344 = ct{1919};
t3440 = ct{1920};
t3441 = ct{1921};
t3442 = ct{1922};
t3443 = ct{1923};
t3444 = ct{1924};
t3445 = ct{1925};
t3446 = ct{1926};
t3447 = ct{1927};
t3448 = ct{1928};
t3449 = ct{1929};
t3450 = ct{1930};
t3453 = ct{1931};
t3454 = ct{1932};
t3455 = ct{1933};
t3456 = ct{1934};
t3457 = ct{1935};
t3458 = ct{1936};
t346 = ct{1937};
t3460 = ct{1938};
t3461 = ct{1939};
t3462 = ct{1940};
t3463 = ct{1941};
t3464 = ct{1942};
t3465 = ct{1943};
t3466 = ct{1944};
t3467 = ct{1945};
t3468 = ct{1946};
t3469 = ct{1947};
t347 = ct{1948};
t3470 = ct{1949};
t3471 = ct{1950};
t3472 = ct{1951};
t3473 = ct{1952};
t3474 = ct{1953};
t3475 = ct{1954};
t3476 = ct{1955};
t3479 = ct{1956};
t348 = ct{1957};
t3480 = ct{1958};
t3481 = ct{1959};
t3483 = ct{1960};
t3484 = ct{1961};
t3485 = ct{1962};
t3487 = ct{1963};
t3488 = ct{1964};
t3489 = ct{1965};
t349 = ct{1966};
t3490 = ct{1967};
t3491 = ct{1968};
t3492 = ct{1969};
t3493 = ct{1970};
t3494 = ct{1971};
t3496 = ct{1972};
t3497 = ct{1973};
t3498 = ct{1974};
t3499 = ct{1975};
t350 = ct{1976};
t3500 = ct{1977};
t3501 = ct{1978};
t3502 = ct{1979};
t3503 = ct{1980};
t3504 = ct{1981};
t3505 = ct{1982};
t3506 = ct{1983};
t3507 = ct{1984};
t3509 = ct{1985};
t3510 = ct{1986};
t3511 = ct{1987};
t3513 = ct{1988};
t3514 = ct{1989};
t3515 = ct{1990};
t3516 = ct{1991};
t3517 = ct{1992};
t3518 = ct{1993};
t352 = ct{1994};
t3521 = ct{1995};
t3522 = ct{1996};
t3523 = ct{1997};
t3526 = ct{1998};
t3529 = ct{1999};
t353 = ct{2000};
t3530 = ct{2001};
t3531 = ct{2002};
t3532 = ct{2003};
t3533 = ct{2004};
t3535 = ct{2005};
t3536 = ct{2006};
t3538 = ct{2007};
t3539 = ct{2008};
t3540 = ct{2009};
t3542 = ct{2010};
t3543 = ct{2011};
t3544 = ct{2012};
t3546 = ct{2013};
t3547 = ct{2014};
t3549 = ct{2015};
t3551 = ct{2016};
t3552 = ct{2017};
t3554 = ct{2018};
t3556 = ct{2019};
t3557 = ct{2020};
t3559 = ct{2021};
t356 = ct{2022};
t3560 = ct{2023};
t3562 = ct{2024};
t3563 = ct{2025};
t3564 = ct{2026};
t3565 = ct{2027};
t3566 = ct{2028};
t3568 = ct{2029};
t3569 = ct{2030};
t357 = ct{2031};
t3570 = ct{2032};
t3571 = ct{2033};
t3572 = ct{2034};
t3573 = ct{2035};
t3574 = ct{2036};
t3577 = ct{2037};
t3578 = ct{2038};
t358 = ct{2039};
t3582 = ct{2040};
t3583 = ct{2041};
t3584 = ct{2042};
t3585 = ct{2043};
t3586 = ct{2044};
t3587 = ct{2045};
t3588 = ct{2046};
t3589 = ct{2047};
t359 = ct{2048};
t3590 = ct{2049};
t3591 = ct{2050};
t3592 = ct{2051};
t3593 = ct{2052};
t3595 = ct{2053};
t3596 = ct{2054};
t3597 = ct{2055};
t3598 = ct{2056};
t3599 = ct{2057};
t3600 = ct{2058};
t3602 = ct{2059};
t3603 = ct{2060};
t3604 = ct{2061};
t3605 = ct{2062};
t3606 = ct{2063};
t3607 = ct{2064};
t3609 = ct{2065};
t361 = ct{2066};
t3610 = ct{2067};
t3611 = ct{2068};
t3612 = ct{2069};
t3616 = ct{2070};
t3617 = ct{2071};
t3618 = ct{2072};
t362 = ct{2073};
t3624 = ct{2074};
t3625 = ct{2075};
t3627 = ct{2076};
t3628 = ct{2077};
t3630 = ct{2078};
t3631 = ct{2079};
t3633 = ct{2080};
t3634 = ct{2081};
t3635 = ct{2082};
t3636 = ct{2083};
t3637 = ct{2084};
t3638 = ct{2085};
t3640 = ct{2086};
t3642 = ct{2087};
t3644 = ct{2088};
t3648 = ct{2089};
t365 = ct{2090};
t3652 = ct{2091};
t3653 = ct{2092};
t3654 = ct{2093};
t3655 = ct{2094};
t3656 = ct{2095};
t3657 = ct{2096};
t3658 = ct{2097};
t3659 = ct{2098};
t3660 = ct{2099};
t3662 = ct{2100};
t3663 = ct{2101};
t3664 = ct{2102};
t3665 = ct{2103};
t3666 = ct{2104};
t3667 = ct{2105};
t3668 = ct{2106};
t3669 = ct{2107};
t3670 = ct{2108};
t3671 = ct{2109};
t3672 = ct{2110};
t3673 = ct{2111};
t3674 = ct{2112};
t3675 = ct{2113};
t3676 = ct{2114};
t3677 = ct{2115};
t3678 = ct{2116};
t3679 = ct{2117};
t368 = ct{2118};
t3681 = ct{2119};
t3682 = ct{2120};
t3683 = ct{2121};
t3684 = ct{2122};
t3687 = ct{2123};
t3689 = ct{2124};
t369 = ct{2125};
t3690 = ct{2126};
t3691 = ct{2127};
t3692 = ct{2128};
t3693 = ct{2129};
t3694 = ct{2130};
t3695 = ct{2131};
t3696 = ct{2132};
t3697 = ct{2133};
t3698 = ct{2134};
t3699 = ct{2135};
t3700 = ct{2136};
t3701 = ct{2137};
t3702 = ct{2138};
t3703 = ct{2139};
t3704 = ct{2140};
t3705 = ct{2141};
t3706 = ct{2142};
t3707 = ct{2143};
t3708 = ct{2144};
t3709 = ct{2145};
t371 = ct{2146};
t3711 = ct{2147};
t3712 = ct{2148};
t3713 = ct{2149};
t3715 = ct{2150};
t3716 = ct{2151};
t3717 = ct{2152};
t3718 = ct{2153};
t3719 = ct{2154};
t372 = ct{2155};
t3720 = ct{2156};
t3724 = ct{2157};
t3725 = ct{2158};
t3726 = ct{2159};
t3727 = ct{2160};
t3728 = ct{2161};
t3729 = ct{2162};
t373 = ct{2163};
t3730 = ct{2164};
t3731 = ct{2165};
t3732 = ct{2166};
t3733 = ct{2167};
t3734 = ct{2168};
t3735 = ct{2169};
t3736 = ct{2170};
t3737 = ct{2171};
t3738 = ct{2172};
t374 = ct{2173};
t3740 = ct{2174};
t3742 = ct{2175};
t3743 = ct{2176};
t3744 = ct{2177};
t3745 = ct{2178};
t3746 = ct{2179};
t3747 = ct{2180};
t3750 = ct{2181};
t3752 = ct{2182};
t3753 = ct{2183};
t3754 = ct{2184};
t3755 = ct{2185};
t3756 = ct{2186};
t3757 = ct{2187};
t3758 = ct{2188};
t3759 = ct{2189};
t3760 = ct{2190};
t3761 = ct{2191};
t3762 = ct{2192};
t3763 = ct{2193};
t3764 = ct{2194};
t3765 = ct{2195};
t3766 = ct{2196};
t3767 = ct{2197};
t3768 = ct{2198};
t3769 = ct{2199};
t377 = ct{2200};
t3772 = ct{2201};
t3774 = ct{2202};
t3777 = ct{2203};
t3778 = ct{2204};
t3779 = ct{2205};
t378 = ct{2206};
t3780 = ct{2207};
t3781 = ct{2208};
t3782 = ct{2209};
t3783 = ct{2210};
t3784 = ct{2211};
t3785 = ct{2212};
t3786 = ct{2213};
t3787 = ct{2214};
t3788 = ct{2215};
t3789 = ct{2216};
t379 = ct{2217};
t3790 = ct{2218};
t3791 = ct{2219};
t3792 = ct{2220};
t3793 = ct{2221};
t3794 = ct{2222};
t3795 = ct{2223};
t3796 = ct{2224};
t3797 = ct{2225};
t3798 = ct{2226};
t3799 = ct{2227};
t380 = ct{2228};
t3800 = ct{2229};
t3807 = ct{2230};
t3808 = ct{2231};
t3809 = ct{2232};
t3810 = ct{2233};
t3811 = ct{2234};
t3812 = ct{2235};
t3813 = ct{2236};
t3814 = ct{2237};
t3815 = ct{2238};
t3816 = ct{2239};
t3817 = ct{2240};
t3818 = ct{2241};
t3819 = ct{2242};
t382 = ct{2243};
t3820 = ct{2244};
t3821 = ct{2245};
t3822 = ct{2246};
t3823 = ct{2247};
t3824 = ct{2248};
t3825 = ct{2249};
t3830 = ct{2250};
t3831 = ct{2251};
t3833 = ct{2252};
t3834 = ct{2253};
t3835 = ct{2254};
t3836 = ct{2255};
t3838 = ct{2256};
t3839 = ct{2257};
t384 = ct{2258};
t3840 = ct{2259};
t3841 = ct{2260};
t3842 = ct{2261};
t3843 = ct{2262};
t3844 = ct{2263};
t3845 = ct{2264};
t3848 = ct{2265};
t3849 = ct{2266};
t3850 = ct{2267};
t3851 = ct{2268};
t3852 = ct{2269};
t3853 = ct{2270};
t3855 = ct{2271};
t3859 = ct{2272};
t386 = ct{2273};
t3861 = ct{2274};
t3862 = ct{2275};
t3863 = ct{2276};
t3864 = ct{2277};
t3865 = ct{2278};
t3866 = ct{2279};
t3868 = ct{2280};
t3869 = ct{2281};
t387 = ct{2282};
t3870 = ct{2283};
t3871 = ct{2284};
t3872 = ct{2285};
t3873 = ct{2286};
t3874 = ct{2287};
t3875 = ct{2288};
t3876 = ct{2289};
t3877 = ct{2290};
t3879 = ct{2291};
t388 = ct{2292};
t3880 = ct{2293};
t3881 = ct{2294};
t3882 = ct{2295};
t3883 = ct{2296};
t3884 = ct{2297};
t3885 = ct{2298};
t3886 = ct{2299};
t3888 = ct{2300};
t3889 = ct{2301};
t3890 = ct{2302};
t3891 = ct{2303};
t3892 = ct{2304};
t3893 = ct{2305};
t3894 = ct{2306};
t3895 = ct{2307};
t3896 = ct{2308};
t3897 = ct{2309};
t3899 = ct{2310};
t3900 = ct{2311};
t3904 = ct{2312};
t3905 = ct{2313};
t3906 = ct{2314};
t3907 = ct{2315};
t3908 = ct{2316};
t3909 = ct{2317};
t391 = ct{2318};
t3910 = ct{2319};
t3911 = ct{2320};
t3912 = ct{2321};
t3913 = ct{2322};
t3914 = ct{2323};
t3915 = ct{2324};
t3916 = ct{2325};
t3917 = ct{2326};
t3918 = ct{2327};
t3919 = ct{2328};
t392 = ct{2329};
t3920 = ct{2330};
t3921 = ct{2331};
t3922 = ct{2332};
t3923 = ct{2333};
t3924 = ct{2334};
t3925 = ct{2335};
t3926 = ct{2336};
t3927 = ct{2337};
t3928 = ct{2338};
t3931 = ct{2339};
t3936 = ct{2340};
t3940 = ct{2341};
t3941 = ct{2342};
t3942 = ct{2343};
t3943 = ct{2344};
t3944 = ct{2345};
t3946 = ct{2346};
t3948 = ct{2347};
t395 = ct{2348};
t3950 = ct{2349};
t3951 = ct{2350};
t3952 = ct{2351};
t3953 = ct{2352};
t3954 = ct{2353};
t3955 = ct{2354};
t3956 = ct{2355};
t3957 = ct{2356};
t3958 = ct{2357};
t3959 = ct{2358};
t396 = ct{2359};
t3960 = ct{2360};
t3961 = ct{2361};
t3962 = ct{2362};
t3963 = ct{2363};
t3964 = ct{2364};
t3965 = ct{2365};
t3966 = ct{2366};
t3967 = ct{2367};
t3968 = ct{2368};
t3969 = ct{2369};
t3971 = ct{2370};
t3972 = ct{2371};
t3973 = ct{2372};
t3974 = ct{2373};
t3975 = ct{2374};
t3976 = ct{2375};
t3977 = ct{2376};
t3978 = ct{2377};
t3979 = ct{2378};
t3982 = ct{2379};
t3983 = ct{2380};
t3984 = ct{2381};
t3985 = ct{2382};
t3986 = ct{2383};
t3987 = ct{2384};
t3988 = ct{2385};
t3989 = ct{2386};
t3994 = ct{2387};
t3995 = ct{2388};
t3996 = ct{2389};
t3997 = ct{2390};
t4 = ct{2391};
t400 = ct{2392};
t4000 = ct{2393};
t4003 = ct{2394};
t4004 = ct{2395};
t4006 = ct{2396};
t4008 = ct{2397};
t4009 = ct{2398};
t401 = ct{2399};
t4010 = ct{2400};
t4011 = ct{2401};
t4012 = ct{2402};
t4013 = ct{2403};
t4014 = ct{2404};
t4015 = ct{2405};
t4016 = ct{2406};
t4017 = ct{2407};
t4018 = ct{2408};
t4019 = ct{2409};
t402 = ct{2410};
t4020 = ct{2411};
t4022 = ct{2412};
t4023 = ct{2413};
t4024 = ct{2414};
t4025 = ct{2415};
t4026 = ct{2416};
t4028 = ct{2417};
t4029 = ct{2418};
t403 = ct{2419};
t4034 = ct{2420};
t4035 = ct{2421};
t4037 = ct{2422};
t4038 = ct{2423};
t4039 = ct{2424};
t4040 = ct{2425};
t4041 = ct{2426};
t4042 = ct{2427};
t4045 = ct{2428};
t4046 = ct{2429};
t4047 = ct{2430};
t4048 = ct{2431};
t4049 = ct{2432};
t4050 = ct{2433};
t4051 = ct{2434};
t4053 = ct{2435};
t4054 = ct{2436};
t4055 = ct{2437};
t4056 = ct{2438};
t4057 = ct{2439};
t4059 = ct{2440};
t406 = ct{2441};
t4060 = ct{2442};
t4061 = ct{2443};
t4062 = ct{2444};
t4063 = ct{2445};
t4064 = ct{2446};
t4065 = ct{2447};
t4066 = ct{2448};
t4067 = ct{2449};
t4068 = ct{2450};
t4069 = ct{2451};
t4070 = ct{2452};
t4071 = ct{2453};
t4073 = ct{2454};
t4074 = ct{2455};
t4075 = ct{2456};
t4079 = ct{2457};
t4080 = ct{2458};
t4081 = ct{2459};
t4082 = ct{2460};
t4083 = ct{2461};
t4084 = ct{2462};
t4085 = ct{2463};
t4086 = ct{2464};
t4087 = ct{2465};
t4089 = ct{2466};
t4090 = ct{2467};
t4091 = ct{2468};
t4092 = ct{2469};
t4093 = ct{2470};
t4094 = ct{2471};
t4095 = ct{2472};
t4097 = ct{2473};
t4098 = ct{2474};
t4099 = ct{2475};
t410 = ct{2476};
t4100 = ct{2477};
t4103 = ct{2478};
t4105 = ct{2479};
t4106 = ct{2480};
t4108 = ct{2481};
t4109 = ct{2482};
t411 = ct{2483};
t4110 = ct{2484};
t4111 = ct{2485};
t4112 = ct{2486};
t4113 = ct{2487};
t4114 = ct{2488};
t4115 = ct{2489};
t4116 = ct{2490};
t4118 = ct{2491};
t4119 = ct{2492};
t412 = ct{2493};
t4120 = ct{2494};
t4123 = ct{2495};
t4124 = ct{2496};
t4125 = ct{2497};
t4126 = ct{2498};
t4127 = ct{2499};
t4128 = ct{2500};
t4129 = ct{2501};
t413 = ct{2502};
t4130 = ct{2503};
t4132 = ct{2504};
t4133 = ct{2505};
t4134 = ct{2506};
t4135 = ct{2507};
t4136 = ct{2508};
t4139 = ct{2509};
t414 = ct{2510};
t4140 = ct{2511};
t4141 = ct{2512};
t4142 = ct{2513};
t4143 = ct{2514};
t4144 = ct{2515};
t4145 = ct{2516};
t4147 = ct{2517};
t4148 = ct{2518};
t4149 = ct{2519};
t415 = ct{2520};
t4151 = ct{2521};
t4152 = ct{2522};
t4153 = ct{2523};
t4154 = ct{2524};
t416 = ct{2525};
t4161 = ct{2526};
t4162 = ct{2527};
t4164 = ct{2528};
t4165 = ct{2529};
t4166 = ct{2530};
t4169 = ct{2531};
t417 = ct{2532};
t4171 = ct{2533};
t4173 = ct{2534};
t4174 = ct{2535};
t4177 = ct{2536};
t4178 = ct{2537};
t4179 = ct{2538};
t418 = ct{2539};
t4180 = ct{2540};
t4181 = ct{2541};
t4183 = ct{2542};
t4184 = ct{2543};
t4185 = ct{2544};
t4186 = ct{2545};
t4188 = ct{2546};
t4190 = ct{2547};
t4195 = ct{2548};
t4196 = ct{2549};
t4197 = ct{2550};
t420 = ct{2551};
t4201 = ct{2552};
t4202 = ct{2553};
t4205 = ct{2554};
t4206 = ct{2555};
t4207 = ct{2556};
t4208 = ct{2557};
t4209 = ct{2558};
t4210 = ct{2559};
t4211 = ct{2560};
t4215 = ct{2561};
t4217 = ct{2562};
t4218 = ct{2563};
t4219 = ct{2564};
t422 = ct{2565};
t4220 = ct{2566};
t4221 = ct{2567};
t4223 = ct{2568};
t4224 = ct{2569};
t4225 = ct{2570};
t4226 = ct{2571};
t4228 = ct{2572};
t4229 = ct{2573};
t423 = ct{2574};
t4230 = ct{2575};
t4231 = ct{2576};
t4232 = ct{2577};
t4233 = ct{2578};
t4234 = ct{2579};
t4235 = ct{2580};
t424 = ct{2581};
t4241 = ct{2582};
t4242 = ct{2583};
t4243 = ct{2584};
t4244 = ct{2585};
t4245 = ct{2586};
t4246 = ct{2587};
t4247 = ct{2588};
t4248 = ct{2589};
t4249 = ct{2590};
t425 = ct{2591};
t4250 = ct{2592};
t4251 = ct{2593};
t4253 = ct{2594};
t4254 = ct{2595};
t4255 = ct{2596};
t4256 = ct{2597};
t4257 = ct{2598};
t4258 = ct{2599};
t4259 = ct{2600};
t4260 = ct{2601};
t4261 = ct{2602};
t4262 = ct{2603};
t4263 = ct{2604};
t427 = ct{2605};
t4273 = ct{2606};
t4274 = ct{2607};
t4275 = ct{2608};
t4276 = ct{2609};
t4278 = ct{2610};
t4279 = ct{2611};
t428 = ct{2612};
t4280 = ct{2613};
t4281 = ct{2614};
t4282 = ct{2615};
t4283 = ct{2616};
t4284 = ct{2617};
t4285 = ct{2618};
t4286 = ct{2619};
t4287 = ct{2620};
t4289 = ct{2621};
t429 = ct{2622};
t4290 = ct{2623};
t4291 = ct{2624};
t4292 = ct{2625};
t4293 = ct{2626};
t4295 = ct{2627};
t4296 = ct{2628};
t4297 = ct{2629};
t4298 = ct{2630};
t4299 = ct{2631};
t4300 = ct{2632};
t4301 = ct{2633};
t4302 = ct{2634};
t4303 = ct{2635};
t4304 = ct{2636};
t4305 = ct{2637};
t4306 = ct{2638};
t4308 = ct{2639};
t431 = ct{2640};
t4310 = ct{2641};
t4315 = ct{2642};
t4316 = ct{2643};
t4317 = ct{2644};
t4318 = ct{2645};
t432 = ct{2646};
t4321 = ct{2647};
t4323 = ct{2648};
t4324 = ct{2649};
t4325 = ct{2650};
t4326 = ct{2651};
t4327 = ct{2652};
t4328 = ct{2653};
t4329 = ct{2654};
t433 = ct{2655};
t4330 = ct{2656};
t4331 = ct{2657};
t4332 = ct{2658};
t4333 = ct{2659};
t4334 = ct{2660};
t4335 = ct{2661};
t4336 = ct{2662};
t4337 = ct{2663};
t4338 = ct{2664};
t4339 = ct{2665};
t434 = ct{2666};
t4340 = ct{2667};
t4342 = ct{2668};
t4344 = ct{2669};
t4345 = ct{2670};
t4346 = ct{2671};
t4347 = ct{2672};
t4348 = ct{2673};
t4349 = ct{2674};
t435 = ct{2675};
t4350 = ct{2676};
t4354 = ct{2677};
t4356 = ct{2678};
t4357 = ct{2679};
t436 = ct{2680};
t4362 = ct{2681};
t4363 = ct{2682};
t4365 = ct{2683};
t4366 = ct{2684};
t4368 = ct{2685};
t4369 = ct{2686};
t437 = ct{2687};
t4370 = ct{2688};
t4371 = ct{2689};
t4372 = ct{2690};
t4373 = ct{2691};
t4374 = ct{2692};
t4375 = ct{2693};
t4376 = ct{2694};
t4377 = ct{2695};
t4378 = ct{2696};
t4379 = ct{2697};
t438 = ct{2698};
t4380 = ct{2699};
t4382 = ct{2700};
t4383 = ct{2701};
t4384 = ct{2702};
t4385 = ct{2703};
t4386 = ct{2704};
t4387 = ct{2705};
t4388 = ct{2706};
t4389 = ct{2707};
t439 = ct{2708};
t4391 = ct{2709};
t4392 = ct{2710};
t4394 = ct{2711};
t4395 = ct{2712};
t4396 = ct{2713};
t4397 = ct{2714};
t4398 = ct{2715};
t4399 = ct{2716};
t44 = ct{2717};
t440 = ct{2718};
t4400 = ct{2719};
t4401 = ct{2720};
t4402 = ct{2721};
t4403 = ct{2722};
t4404 = ct{2723};
t4405 = ct{2724};
t4406 = ct{2725};
t4407 = ct{2726};
t4408 = ct{2727};
t4409 = ct{2728};
t441 = ct{2729};
t4410 = ct{2730};
t4411 = ct{2731};
t4412 = ct{2732};
t4413 = ct{2733};
t4414 = ct{2734};
t4415 = ct{2735};
t4416 = ct{2736};
t4417 = ct{2737};
t4418 = ct{2738};
t4419 = ct{2739};
t442 = ct{2740};
t4420 = ct{2741};
t4421 = ct{2742};
t4422 = ct{2743};
t4423 = ct{2744};
t4424 = ct{2745};
t4425 = ct{2746};
t4426 = ct{2747};
t4427 = ct{2748};
t4428 = ct{2749};
t4429 = ct{2750};
t4430 = ct{2751};
t4431 = ct{2752};
t4432 = ct{2753};
t4433 = ct{2754};
t4434 = ct{2755};
t4435 = ct{2756};
t4436 = ct{2757};
t4437 = ct{2758};
t4438 = ct{2759};
t4439 = ct{2760};
t444 = ct{2761};
t4440 = ct{2762};
t4442 = ct{2763};
t4444 = ct{2764};
t4445 = ct{2765};
t4446 = ct{2766};
t4447 = ct{2767};
t4448 = ct{2768};
t4449 = ct{2769};
t445 = ct{2770};
t4450 = ct{2771};
t4451 = ct{2772};
t4453 = ct{2773};
t4454 = ct{2774};
t4455 = ct{2775};
t4460 = ct{2776};
t4461 = ct{2777};
t4462 = ct{2778};
t4463 = ct{2779};
t4464 = ct{2780};
t4465 = ct{2781};
t4466 = ct{2782};
t4467 = ct{2783};
t4468 = ct{2784};
t4469 = ct{2785};
t4470 = ct{2786};
t4471 = ct{2787};
t4473 = ct{2788};
t4474 = ct{2789};
t4475 = ct{2790};
t4476 = ct{2791};
t4477 = ct{2792};
t4478 = ct{2793};
t4479 = ct{2794};
t448 = ct{2795};
t4481 = ct{2796};
t4482 = ct{2797};
t4483 = ct{2798};
t4484 = ct{2799};
t4485 = ct{2800};
t4486 = ct{2801};
t4487 = ct{2802};
t4488 = ct{2803};
t4489 = ct{2804};
t449 = ct{2805};
t4490 = ct{2806};
t4493 = ct{2807};
t4494 = ct{2808};
t4495 = ct{2809};
t4496 = ct{2810};
t4497 = ct{2811};
t4498 = ct{2812};
t4499 = ct{2813};
t45 = ct{2814};
t450 = ct{2815};
t4500 = ct{2816};
t4501 = ct{2817};
t4502 = ct{2818};
t4503 = ct{2819};
t4504 = ct{2820};
t4505 = ct{2821};
t4506 = ct{2822};
t4507 = ct{2823};
t4508 = ct{2824};
t4509 = ct{2825};
t4510 = ct{2826};
t4512 = ct{2827};
t4513 = ct{2828};
t4514 = ct{2829};
t4515 = ct{2830};
t4516 = ct{2831};
t4518 = ct{2832};
t4519 = ct{2833};
t452 = ct{2834};
t4520 = ct{2835};
t4521 = ct{2836};
t4522 = ct{2837};
t4523 = ct{2838};
t4524 = ct{2839};
t4525 = ct{2840};
t4526 = ct{2841};
t4527 = ct{2842};
t4529 = ct{2843};
t453 = ct{2844};
t4530 = ct{2845};
t4531 = ct{2846};
t4532 = ct{2847};
t4534 = ct{2848};
t4535 = ct{2849};
t4536 = ct{2850};
t4537 = ct{2851};
t4538 = ct{2852};
t4539 = ct{2853};
t454 = ct{2854};
t4541 = ct{2855};
t4543 = ct{2856};
t4544 = ct{2857};
t4545 = ct{2858};
t4546 = ct{2859};
t4547 = ct{2860};
t4549 = ct{2861};
t4550 = ct{2862};
t4551 = ct{2863};
t4552 = ct{2864};
t4553 = ct{2865};
t4554 = ct{2866};
t4556 = ct{2867};
t4557 = ct{2868};
t4558 = ct{2869};
t4559 = ct{2870};
t4560 = ct{2871};
t4564 = ct{2872};
t4565 = ct{2873};
t4566 = ct{2874};
t4567 = ct{2875};
t4568 = ct{2876};
t4569 = ct{2877};
t457 = ct{2878};
t4570 = ct{2879};
t4572 = ct{2880};
t4573 = ct{2881};
t4575 = ct{2882};
t4576 = ct{2883};
t4577 = ct{2884};
t4578 = ct{2885};
t458 = ct{2886};
t4580 = ct{2887};
t4581 = ct{2888};
t4582 = ct{2889};
t4584 = ct{2890};
t4585 = ct{2891};
t4586 = ct{2892};
t4587 = ct{2893};
t4588 = ct{2894};
t4589 = ct{2895};
t459 = ct{2896};
t4590 = ct{2897};
t4591 = ct{2898};
t4592 = ct{2899};
t4593 = ct{2900};
t4594 = ct{2901};
t4595 = ct{2902};
t4596 = ct{2903};
t4597 = ct{2904};
t4598 = ct{2905};
t4599 = ct{2906};
t46 = ct{2907};
t460 = ct{2908};
t4600 = ct{2909};
t4601 = ct{2910};
t4602 = ct{2911};
t4603 = ct{2912};
t4604 = ct{2913};
t4605 = ct{2914};
t4606 = ct{2915};
t4607 = ct{2916};
t4608 = ct{2917};
t4609 = ct{2918};
t461 = ct{2919};
t4610 = ct{2920};
t4612 = ct{2921};
t4613 = ct{2922};
t4614 = ct{2923};
t4615 = ct{2924};
t4616 = ct{2925};
t4617 = ct{2926};
t4618 = ct{2927};
t4619 = ct{2928};
t462 = ct{2929};
t4620 = ct{2930};
t4621 = ct{2931};
t4622 = ct{2932};
t4623 = ct{2933};
t4624 = ct{2934};
t4625 = ct{2935};
t4626 = ct{2936};
t4627 = ct{2937};
t4629 = ct{2938};
t463 = ct{2939};
t4631 = ct{2940};
t4632 = ct{2941};
t4633 = ct{2942};
t4634 = ct{2943};
t4635 = ct{2944};
t4636 = ct{2945};
t4637 = ct{2946};
t4638 = ct{2947};
t4639 = ct{2948};
t464 = ct{2949};
t4640 = ct{2950};
t4643 = ct{2951};
t4644 = ct{2952};
t4645 = ct{2953};
t4646 = ct{2954};
t4647 = ct{2955};
t4648 = ct{2956};
t4649 = ct{2957};
t465 = ct{2958};
t4650 = ct{2959};
t4652 = ct{2960};
t4653 = ct{2961};
t4654 = ct{2962};
t4655 = ct{2963};
t4656 = ct{2964};
t4657 = ct{2965};
t4659 = ct{2966};
t466 = ct{2967};
t4660 = ct{2968};
t4661 = ct{2969};
t4662 = ct{2970};
t4663 = ct{2971};
t4664 = ct{2972};
t4665 = ct{2973};
t4666 = ct{2974};
t4667 = ct{2975};
t4668 = ct{2976};
t4669 = ct{2977};
t4670 = ct{2978};
t4671 = ct{2979};
t4672 = ct{2980};
t4673 = ct{2981};
t4674 = ct{2982};
t4675 = ct{2983};
t4676 = ct{2984};
t4677 = ct{2985};
t4678 = ct{2986};
t4679 = ct{2987};
t468 = ct{2988};
t4680 = ct{2989};
t4681 = ct{2990};
t4682 = ct{2991};
t4683 = ct{2992};
t4684 = ct{2993};
t4685 = ct{2994};
t4686 = ct{2995};
t4687 = ct{2996};
t4689 = ct{2997};
t469 = ct{2998};
t4692 = ct{2999};
t4693 = ct{3000};
t4694 = ct{3001};
t4695 = ct{3002};
t4696 = ct{3003};
t4697 = ct{3004};
t4698 = ct{3005};
t4699 = ct{3006};
t47 = ct{3007};
t470 = ct{3008};
t4700 = ct{3009};
t4702 = ct{3010};
t4703 = ct{3011};
t4704 = ct{3012};
t4707 = ct{3013};
t4708 = ct{3014};
t4709 = ct{3015};
t471 = ct{3016};
t4710 = ct{3017};
t4711 = ct{3018};
t4712 = ct{3019};
t4713 = ct{3020};
t4714 = ct{3021};
t4715 = ct{3022};
t4716 = ct{3023};
t4717 = ct{3024};
t4718 = ct{3025};
t4719 = ct{3026};
t472 = ct{3027};
t4720 = ct{3028};
t4721 = ct{3029};
t4722 = ct{3030};
t4723 = ct{3031};
t4724 = ct{3032};
t4725 = ct{3033};
t4726 = ct{3034};
t4727 = ct{3035};
t4728 = ct{3036};
t4729 = ct{3037};
t4730 = ct{3038};
t4731 = ct{3039};
t4732 = ct{3040};
t4733 = ct{3041};
t4734 = ct{3042};
t4736 = ct{3043};
t4737 = ct{3044};
t4738 = ct{3045};
t4739 = ct{3046};
t4740 = ct{3047};
t4742 = ct{3048};
t4745 = ct{3049};
t4746 = ct{3050};
t4747 = ct{3051};
t4748 = ct{3052};
t475 = ct{3053};
t4750 = ct{3054};
t4751 = ct{3055};
t4753 = ct{3056};
t4754 = ct{3057};
t4755 = ct{3058};
t4756 = ct{3059};
t4757 = ct{3060};
t4762 = ct{3061};
t4763 = ct{3062};
t4765 = ct{3063};
t4768 = ct{3064};
t477 = ct{3065};
t4771 = ct{3066};
t4772 = ct{3067};
t4773 = ct{3068};
t4774 = ct{3069};
t4775 = ct{3070};
t4776 = ct{3071};
t4779 = ct{3072};
t4780 = ct{3073};
t4781 = ct{3074};
t4782 = ct{3075};
t4783 = ct{3076};
t4784 = ct{3077};
t4785 = ct{3078};
t4786 = ct{3079};
t4787 = ct{3080};
t4788 = ct{3081};
t4789 = ct{3082};
t479 = ct{3083};
t4790 = ct{3084};
t4791 = ct{3085};
t4792 = ct{3086};
t4793 = ct{3087};
t4794 = ct{3088};
t4795 = ct{3089};
t4797 = ct{3090};
t4799 = ct{3091};
t480 = ct{3092};
t4800 = ct{3093};
t4801 = ct{3094};
t4802 = ct{3095};
t4803 = ct{3096};
t4805 = ct{3097};
t4806 = ct{3098};
t4809 = ct{3099};
t481 = ct{3100};
t4810 = ct{3101};
t4811 = ct{3102};
t4812 = ct{3103};
t4813 = ct{3104};
t4814 = ct{3105};
t4816 = ct{3106};
t4817 = ct{3107};
t4818 = ct{3108};
t4819 = ct{3109};
t482 = ct{3110};
t4820 = ct{3111};
t4822 = ct{3112};
t4823 = ct{3113};
t4824 = ct{3114};
t4825 = ct{3115};
t4826 = ct{3116};
t4827 = ct{3117};
t4829 = ct{3118};
t483 = ct{3119};
t4831 = ct{3120};
t4833 = ct{3121};
t4834 = ct{3122};
t4835 = ct{3123};
t4837 = ct{3124};
t484 = ct{3125};
t4840 = ct{3126};
t4841 = ct{3127};
t4842 = ct{3128};
t4843 = ct{3129};
t4844 = ct{3130};
t4845 = ct{3131};
t4846 = ct{3132};
t4848 = ct{3133};
t485 = ct{3134};
t4850 = ct{3135};
t4853 = ct{3136};
t4854 = ct{3137};
t4855 = ct{3138};
t4856 = ct{3139};
t4857 = ct{3140};
t4858 = ct{3141};
t4859 = ct{3142};
t486 = ct{3143};
t4862 = ct{3144};
t4863 = ct{3145};
t4864 = ct{3146};
t4865 = ct{3147};
t4866 = ct{3148};
t4867 = ct{3149};
t4868 = ct{3150};
t4869 = ct{3151};
t4870 = ct{3152};
t4872 = ct{3153};
t4873 = ct{3154};
t4874 = ct{3155};
t4875 = ct{3156};
t4876 = ct{3157};
t4877 = ct{3158};
t488 = ct{3159};
t4880 = ct{3160};
t4881 = ct{3161};
t4884 = ct{3162};
t4888 = ct{3163};
t4889 = ct{3164};
t489 = ct{3165};
t4890 = ct{3166};
t4893 = ct{3167};
t4894 = ct{3168};
t4895 = ct{3169};
t4896 = ct{3170};
t4898 = ct{3171};
t4901 = ct{3172};
t4902 = ct{3173};
t4903 = ct{3174};
t4904 = ct{3175};
t4905 = ct{3176};
t4906 = ct{3177};
t4907 = ct{3178};
t4908 = ct{3179};
t491 = ct{3180};
t4911 = ct{3181};
t4913 = ct{3182};
t4914 = ct{3183};
t4919 = ct{3184};
t492 = ct{3185};
t4920 = ct{3186};
t4922 = ct{3187};
t4924 = ct{3188};
t4925 = ct{3189};
t4927 = ct{3190};
t4928 = ct{3191};
t4929 = ct{3192};
t493 = ct{3193};
t4931 = ct{3194};
t4932 = ct{3195};
t4933 = ct{3196};
t4934 = ct{3197};
t4935 = ct{3198};
t4936 = ct{3199};
t4939 = ct{3200};
t494 = ct{3201};
t4942 = ct{3202};
t4943 = ct{3203};
t4944 = ct{3204};
t4946 = ct{3205};
t4947 = ct{3206};
t4948 = ct{3207};
t4949 = ct{3208};
t4950 = ct{3209};
t4951 = ct{3210};
t4952 = ct{3211};
t4953 = ct{3212};
t4957 = ct{3213};
t4959 = ct{3214};
t496 = ct{3215};
t4960 = ct{3216};
t4961 = ct{3217};
t4963 = ct{3218};
t4964 = ct{3219};
t4965 = ct{3220};
t4966 = ct{3221};
t4967 = ct{3222};
t4969 = ct{3223};
t497 = ct{3224};
t4970 = ct{3225};
t4973 = ct{3226};
t4974 = ct{3227};
t4975 = ct{3228};
t4976 = ct{3229};
t4978 = ct{3230};
t4979 = ct{3231};
t498 = ct{3232};
t4981 = ct{3233};
t4982 = ct{3234};
t4983 = ct{3235};
t4984 = ct{3236};
t4987 = ct{3237};
t4988 = ct{3238};
t4989 = ct{3239};
t499 = ct{3240};
t4990 = ct{3241};
t4991 = ct{3242};
t4992 = ct{3243};
t4993 = ct{3244};
t4994 = ct{3245};
t4995 = ct{3246};
t4996 = ct{3247};
t5 = ct{3248};
t50 = ct{3249};
t500 = ct{3250};
t5000 = ct{3251};
t5001 = ct{3252};
t5002 = ct{3253};
t5003 = ct{3254};
t5005 = ct{3255};
t5006 = ct{3256};
t5007 = ct{3257};
t5008 = ct{3258};
t5009 = ct{3259};
t501 = ct{3260};
t5010 = ct{3261};
t5013 = ct{3262};
t5014 = ct{3263};
t5015 = ct{3264};
t5016 = ct{3265};
t5017 = ct{3266};
t5018 = ct{3267};
t5019 = ct{3268};
t502 = ct{3269};
t5020 = ct{3270};
t5021 = ct{3271};
t5022 = ct{3272};
t5023 = ct{3273};
t5024 = ct{3274};
t5026 = ct{3275};
t5027 = ct{3276};
t5028 = ct{3277};
t5029 = ct{3278};
t503 = ct{3279};
t5031 = ct{3280};
t5032 = ct{3281};
t5035 = ct{3282};
t5036 = ct{3283};
t5037 = ct{3284};
t5039 = ct{3285};
t504 = ct{3286};
t5041 = ct{3287};
t5045 = ct{3288};
t5047 = ct{3289};
t5048 = ct{3290};
t505 = ct{3291};
t5051 = ct{3292};
t5054 = ct{3293};
t5055 = ct{3294};
t5056 = ct{3295};
t5057 = ct{3296};
t5058 = ct{3297};
t5059 = ct{3298};
t506 = ct{3299};
t5061 = ct{3300};
t5063 = ct{3301};
t5064 = ct{3302};
t5065 = ct{3303};
t5066 = ct{3304};
t5067 = ct{3305};
t5068 = ct{3306};
t507 = ct{3307};
t5073 = ct{3308};
t5074 = ct{3309};
t5075 = ct{3310};
t5076 = ct{3311};
t5077 = ct{3312};
t5078 = ct{3313};
t5079 = ct{3314};
t508 = ct{3315};
t5080 = ct{3316};
t5083 = ct{3317};
t5084 = ct{3318};
t5085 = ct{3319};
t5086 = ct{3320};
t5087 = ct{3321};
t5088 = ct{3322};
t5089 = ct{3323};
t509 = ct{3324};
t5090 = ct{3325};
t5091 = ct{3326};
t5092 = ct{3327};
t5093 = ct{3328};
t5094 = ct{3329};
t5095 = ct{3330};
t5097 = ct{3331};
t5098 = ct{3332};
t5099 = ct{3333};
t510 = ct{3334};
t5100 = ct{3335};
t5101 = ct{3336};
t5102 = ct{3337};
t5103 = ct{3338};
t5104 = ct{3339};
t5105 = ct{3340};
t5107 = ct{3341};
t5109 = ct{3342};
t511 = ct{3343};
t5110 = ct{3344};
t5112 = ct{3345};
t5113 = ct{3346};
t5114 = ct{3347};
t5117 = ct{3348};
t5118 = ct{3349};
t5119 = ct{3350};
t512 = ct{3351};
t5120 = ct{3352};
t5121 = ct{3353};
t5123 = ct{3354};
t5124 = ct{3355};
t5126 = ct{3356};
t5128 = ct{3357};
t513 = ct{3358};
t5131 = ct{3359};
t5132 = ct{3360};
t5133 = ct{3361};
t5134 = ct{3362};
t5135 = ct{3363};
t5136 = ct{3364};
t5137 = ct{3365};
t5138 = ct{3366};
t5139 = ct{3367};
t514 = ct{3368};
t5140 = ct{3369};
t5141 = ct{3370};
t5143 = ct{3371};
t5146 = ct{3372};
t5147 = ct{3373};
t5148 = ct{3374};
t5150 = ct{3375};
t5151 = ct{3376};
t5154 = ct{3377};
t5156 = ct{3378};
t5157 = ct{3379};
t5158 = ct{3380};
t5159 = ct{3381};
t516 = ct{3382};
t5160 = ct{3383};
t5162 = ct{3384};
t5164 = ct{3385};
t5166 = ct{3386};
t5167 = ct{3387};
t517 = ct{3388};
t5171 = ct{3389};
t5172 = ct{3390};
t5173 = ct{3391};
t5174 = ct{3392};
t5175 = ct{3393};
t5177 = ct{3394};
t518 = ct{3395};
t5180 = ct{3396};
t5181 = ct{3397};
t5182 = ct{3398};
t5183 = ct{3399};
t5184 = ct{3400};
t5185 = ct{3401};
t5187 = ct{3402};
t5188 = ct{3403};
t5189 = ct{3404};
t5190 = ct{3405};
t5191 = ct{3406};
t5194 = ct{3407};
t5195 = ct{3408};
t5197 = ct{3409};
t5199 = ct{3410};
t520 = ct{3411};
t5200 = ct{3412};
t5201 = ct{3413};
t5202 = ct{3414};
t5203 = ct{3415};
t5204 = ct{3416};
t5205 = ct{3417};
t5206 = ct{3418};
t5207 = ct{3419};
t5209 = ct{3420};
t521 = ct{3421};
t5210 = ct{3422};
t5211 = ct{3423};
t5213 = ct{3424};
t5214 = ct{3425};
t5215 = ct{3426};
t5216 = ct{3427};
t5217 = ct{3428};
t5218 = ct{3429};
t5219 = ct{3430};
t522 = ct{3431};
t5220 = ct{3432};
t5221 = ct{3433};
t5222 = ct{3434};
t5223 = ct{3435};
t5224 = ct{3436};
t5225 = ct{3437};
t5226 = ct{3438};
t5227 = ct{3439};
t5229 = ct{3440};
t523 = ct{3441};
t5233 = ct{3442};
t5236 = ct{3443};
t5237 = ct{3444};
t5238 = ct{3445};
t5239 = ct{3446};
t524 = ct{3447};
t5240 = ct{3448};
t5242 = ct{3449};
t5243 = ct{3450};
t5244 = ct{3451};
t5247 = ct{3452};
t5248 = ct{3453};
t5249 = ct{3454};
t525 = ct{3455};
t5251 = ct{3456};
t5252 = ct{3457};
t5255 = ct{3458};
t5258 = ct{3459};
t526 = ct{3460};
t5261 = ct{3461};
t5262 = ct{3462};
t5265 = ct{3463};
t5268 = ct{3464};
t5269 = ct{3465};
t527 = ct{3466};
t5270 = ct{3467};
t5272 = ct{3468};
t5275 = ct{3469};
t5276 = ct{3470};
t5277 = ct{3471};
t5278 = ct{3472};
t5279 = ct{3473};
t528 = ct{3474};
t5280 = ct{3475};
t5285 = ct{3476};
t5287 = ct{3477};
t5288 = ct{3478};
t529 = ct{3479};
t5291 = ct{3480};
t5292 = ct{3481};
t5293 = ct{3482};
t5294 = ct{3483};
t5295 = ct{3484};
t5297 = ct{3485};
t5298 = ct{3486};
t53 = ct{3487};
t530 = ct{3488};
t5302 = ct{3489};
t5303 = ct{3490};
t5304 = ct{3491};
t5306 = ct{3492};
t5308 = ct{3493};
t531 = ct{3494};
t5310 = ct{3495};
t5317 = ct{3496};
t5318 = ct{3497};
t532 = ct{3498};
t5320 = ct{3499};
t5321 = ct{3500};
t5322 = ct{3501};
t5324 = ct{3502};
t5326 = ct{3503};
t5327 = ct{3504};
t5329 = ct{3505};
t533 = ct{3506};
t5330 = ct{3507};
t5331 = ct{3508};
t5332 = ct{3509};
t5334 = ct{3510};
t5336 = ct{3511};
t5339 = ct{3512};
t534 = ct{3513};
t5341 = ct{3514};
t5344 = ct{3515};
t5346 = ct{3516};
t5347 = ct{3517};
t5348 = ct{3518};
t5349 = ct{3519};
t535 = ct{3520};
t5351 = ct{3521};
t5355 = ct{3522};
t5356 = ct{3523};
t5358 = ct{3524};
t5359 = ct{3525};
t536 = ct{3526};
t5361 = ct{3527};
t5364 = ct{3528};
t5365 = ct{3529};
t5367 = ct{3530};
t5368 = ct{3531};
t537 = ct{3532};
t5372 = ct{3533};
t5373 = ct{3534};
t5374 = ct{3535};
t5375 = ct{3536};
t5378 = ct{3537};
t538 = ct{3538};
t5383 = ct{3539};
t5386 = ct{3540};
t5387 = ct{3541};
t5388 = ct{3542};
t5389 = ct{3543};
t539 = ct{3544};
t5390 = ct{3545};
t5391 = ct{3546};
t5392 = ct{3547};
t5393 = ct{3548};
t5394 = ct{3549};
t5395 = ct{3550};
t540 = ct{3551};
t5402 = ct{3552};
t5404 = ct{3553};
t5406 = ct{3554};
t5408 = ct{3555};
t5409 = ct{3556};
t5411 = ct{3557};
t5416 = ct{3558};
t5420 = ct{3559};
t543 = ct{3560};
t5433 = ct{3561};
t5435 = ct{3562};
t5436 = ct{3563};
t5437 = ct{3564};
t5438 = ct{3565};
t544 = ct{3566};
t5440 = ct{3567};
t5441 = ct{3568};
t5442 = ct{3569};
t5443 = ct{3570};
t5444 = ct{3571};
t5445 = ct{3572};
t5448 = ct{3573};
t545 = ct{3574};
t5450 = ct{3575};
t5451 = ct{3576};
t5453 = ct{3577};
t5454 = ct{3578};
t5457 = ct{3579};
t5459 = ct{3580};
t546 = ct{3581};
t5460 = ct{3582};
t5461 = ct{3583};
t5462 = ct{3584};
t5463 = ct{3585};
t5464 = ct{3586};
t5465 = ct{3587};
t5466 = ct{3588};
t547 = ct{3589};
t5473 = ct{3590};
t5475 = ct{3591};
t5479 = ct{3592};
t548 = ct{3593};
t5480 = ct{3594};
t5481 = ct{3595};
t5482 = ct{3596};
t5483 = ct{3597};
t5484 = ct{3598};
t5485 = ct{3599};
t5486 = ct{3600};
t5487 = ct{3601};
t5488 = ct{3602};
t5489 = ct{3603};
t549 = ct{3604};
t5490 = ct{3605};
t5491 = ct{3606};
t5492 = ct{3607};
t5493 = ct{3608};
t5494 = ct{3609};
t5495 = ct{3610};
t5498 = ct{3611};
t5499 = ct{3612};
t5500 = ct{3613};
t5501 = ct{3614};
t5502 = ct{3615};
t5503 = ct{3616};
t5504 = ct{3617};
t5505 = ct{3618};
t5506 = ct{3619};
t5507 = ct{3620};
t551 = ct{3621};
t5512 = ct{3622};
t5513 = ct{3623};
t5514 = ct{3624};
t5516 = ct{3625};
t5517 = ct{3626};
t5518 = ct{3627};
t5519 = ct{3628};
t552 = ct{3629};
t5520 = ct{3630};
t5521 = ct{3631};
t5523 = ct{3632};
t5524 = ct{3633};
t5525 = ct{3634};
t5526 = ct{3635};
t5528 = ct{3636};
t553 = ct{3637};
t5531 = ct{3638};
t5533 = ct{3639};
t5536 = ct{3640};
t5537 = ct{3641};
t554 = ct{3642};
t5540 = ct{3643};
t5541 = ct{3644};
t5542 = ct{3645};
t5543 = ct{3646};
t5544 = ct{3647};
t5546 = ct{3648};
t5548 = ct{3649};
t5549 = ct{3650};
t555 = ct{3651};
t5550 = ct{3652};
t5551 = ct{3653};
t5552 = ct{3654};
t5553 = ct{3655};
t5554 = ct{3656};
t5555 = ct{3657};
t5556 = ct{3658};
t556 = ct{3659};
t5561 = ct{3660};
t5562 = ct{3661};
t5563 = ct{3662};
t5565 = ct{3663};
t5566 = ct{3664};
t5567 = ct{3665};
t5568 = ct{3666};
t5569 = ct{3667};
t557 = ct{3668};
t5570 = ct{3669};
t5571 = ct{3670};
t5572 = ct{3671};
t5573 = ct{3672};
t5578 = ct{3673};
t558 = ct{3674};
t5580 = ct{3675};
t5581 = ct{3676};
t5583 = ct{3677};
t5584 = ct{3678};
t5585 = ct{3679};
t5587 = ct{3680};
t5588 = ct{3681};
t5589 = ct{3682};
t559 = ct{3683};
t5590 = ct{3684};
t5593 = ct{3685};
t5595 = ct{3686};
t5596 = ct{3687};
t5599 = ct{3688};
t560 = ct{3689};
t5601 = ct{3690};
t5603 = ct{3691};
t5604 = ct{3692};
t5607 = ct{3693};
t5608 = ct{3694};
t5609 = ct{3695};
t561 = ct{3696};
t5610 = ct{3697};
t5612 = ct{3698};
t5613 = ct{3699};
t5614 = ct{3700};
t5616 = ct{3701};
t5618 = ct{3702};
t562 = ct{3703};
t5620 = ct{3704};
t5621 = ct{3705};
t5629 = ct{3706};
t563 = ct{3707};
t5631 = ct{3708};
t5633 = ct{3709};
t5634 = ct{3710};
t5635 = ct{3711};
t5636 = ct{3712};
t564 = ct{3713};
t5658 = ct{3714};
t5664 = ct{3715};
t5665 = ct{3716};
t5669 = ct{3717};
t567 = ct{3718};
t5670 = ct{3719};
t5673 = ct{3720};
t5678 = ct{3721};
t568 = ct{3722};
t5688 = ct{3723};
t569 = ct{3724};
t57 = ct{3725};
t570 = ct{3726};
t571 = ct{3727};
t572 = ct{3728};
t573 = ct{3729};
t574 = ct{3730};
t5741 = ct{3731};
t5743 = ct{3732};
t576 = ct{3733};
t577 = ct{3734};
t5777 = ct{3735};
t5778 = ct{3736};
t5779 = ct{3737};
t578 = ct{3738};
t5780 = ct{3739};
t5781 = ct{3740};
t5782 = ct{3741};
t579 = ct{3742};
t58 = ct{3743};
t580 = ct{3744};
t581 = ct{3745};
t5815 = ct{3746};
t5818 = ct{3747};
t5819 = ct{3748};
t582 = ct{3749};
t5823 = ct{3750};
t5825 = ct{3751};
t5826 = ct{3752};
t583 = ct{3753};
t584 = ct{3754};
t586 = ct{3755};
t587 = ct{3756};
t5886 = ct{3757};
t5887 = ct{3758};
t589 = ct{3759};
t5894 = ct{3760};
t59 = ct{3761};
t590 = ct{3762};
t591 = ct{3763};
t5917 = ct{3764};
t592 = ct{3765};
t593 = ct{3766};
t594 = ct{3767};
t595 = ct{3768};
t5958 = ct{3769};
t596 = ct{3770};
t597 = ct{3771};
t5998 = ct{3772};
t5999 = ct{3773};
t6 = ct{3774};
t60 = ct{3775};
t600 = ct{3776};
t602 = ct{3777};
t603 = ct{3778};
t604 = ct{3779};
t605 = ct{3780};
t609 = ct{3781};
t610 = ct{3782};
t611 = ct{3783};
t612 = ct{3784};
t613 = ct{3785};
t614 = ct{3786};
t615 = ct{3787};
t616 = ct{3788};
t618 = ct{3789};
t619 = ct{3790};
t620 = ct{3791};
t621 = ct{3792};
t622 = ct{3793};
t623 = ct{3794};
t624 = ct{3795};
t625 = ct{3796};
t626 = ct{3797};
t629 = ct{3798};
t632 = ct{3799};
t633 = ct{3800};
t634 = ct{3801};
t638 = ct{3802};
t639 = ct{3803};
t640 = ct{3804};
t641 = ct{3805};
t642 = ct{3806};
t643 = ct{3807};
t645 = ct{3808};
t646 = ct{3809};
t647 = ct{3810};
t648 = ct{3811};
t649 = ct{3812};
t650 = ct{3813};
t653 = ct{3814};
t654 = ct{3815};
t657 = ct{3816};
t658 = ct{3817};
t660 = ct{3818};
t661 = ct{3819};
t662 = ct{3820};
t663 = ct{3821};
t664 = ct{3822};
t665 = ct{3823};
t667 = ct{3824};
t668 = ct{3825};
t669 = ct{3826};
t673 = ct{3827};
t674 = ct{3828};
t675 = ct{3829};
t676 = ct{3830};
t677 = ct{3831};
t679 = ct{3832};
t680 = ct{3833};
t681 = ct{3834};
t682 = ct{3835};
t683 = ct{3836};
t684 = ct{3837};
t685 = ct{3838};
t686 = ct{3839};
t687 = ct{3840};
t688 = ct{3841};
t689 = ct{3842};
t692 = ct{3843};
t693 = ct{3844};
t694 = ct{3845};
t695 = ct{3846};
t696 = ct{3847};
t697 = ct{3848};
t698 = ct{3849};
t7 = ct{3850};
t700 = ct{3851};
t702 = ct{3852};
t703 = ct{3853};
t704 = ct{3854};
t705 = ct{3855};
t706 = ct{3856};
t708 = ct{3857};
t71 = ct{3858};
t710 = ct{3859};
t711 = ct{3860};
t712 = ct{3861};
t713 = ct{3862};
t7148 = ct{3863};
t7149 = ct{3864};
t715 = ct{3865};
t716 = ct{3866};
t72 = ct{3867};
t724 = ct{3868};
t728 = ct{3869};
t729 = ct{3870};
t73 = ct{3871};
t731 = ct{3872};
t733 = ct{3873};
t734 = ct{3874};
t735 = ct{3875};
t736 = ct{3876};
t738 = ct{3877};
t739 = ct{3878};
t74 = ct{3879};
t741 = ct{3880};
t742 = ct{3881};
t743 = ct{3882};
t744 = ct{3883};
t746 = ct{3884};
t747 = ct{3885};
t748 = ct{3886};
t749 = ct{3887};
t75 = ct{3888};
t750 = ct{3889};
t751 = ct{3890};
t752 = ct{3891};
t753 = ct{3892};
t754 = ct{3893};
t755 = ct{3894};
t756 = ct{3895};
t757 = ct{3896};
t758 = ct{3897};
t759 = ct{3898};
t76 = ct{3899};
t760 = ct{3900};
t762 = ct{3901};
t763 = ct{3902};
t764 = ct{3903};
t765 = ct{3904};
t766 = ct{3905};
t767 = ct{3906};
t768 = ct{3907};
t769 = ct{3908};
t77 = ct{3909};
t772 = ct{3910};
t773 = ct{3911};
t774 = ct{3912};
t775 = ct{3913};
t776 = ct{3914};
t777 = ct{3915};
t778 = ct{3916};
t779 = ct{3917};
t780 = ct{3918};
t781 = ct{3919};
t782 = ct{3920};
t784 = ct{3921};
t785 = ct{3922};
t786 = ct{3923};
t792 = ct{3924};
t794 = ct{3925};
t795 = ct{3926};
t796 = ct{3927};
t797 = ct{3928};
t798 = ct{3929};
t799 = ct{3930};
t8 = ct{3931};
t80 = ct{3932};
t801 = ct{3933};
t802 = ct{3934};
t803 = ct{3935};
t804 = ct{3936};
t805 = ct{3937};
t806 = ct{3938};
t808 = ct{3939};
t81 = ct{3940};
t814 = ct{3941};
t815 = ct{3942};
t817 = ct{3943};
t820 = ct{3944};
t822 = ct{3945};
t823 = ct{3946};
t824 = ct{3947};
t825 = ct{3948};
t826 = ct{3949};
t827 = ct{3950};
t829 = ct{3951};
t83 = ct{3952};
t830 = ct{3953};
t831 = ct{3954};
t832 = ct{3955};
t833 = ct{3956};
t834 = ct{3957};
t835 = ct{3958};
t836 = ct{3959};
t837 = ct{3960};
t838 = ct{3961};
t84 = ct{3962};
t840 = ct{3963};
t841 = ct{3964};
t842 = ct{3965};
t843 = ct{3966};
t845 = ct{3967};
t846 = ct{3968};
t847 = ct{3969};
t848 = ct{3970};
t852 = ct{3971};
t853 = ct{3972};
t856 = ct{3973};
t86 = ct{3974};
t861 = ct{3975};
t863 = ct{3976};
t866 = ct{3977};
t868 = ct{3978};
t869 = ct{3979};
t870 = ct{3980};
t874 = ct{3981};
t875 = ct{3982};
t876 = ct{3983};
t877 = ct{3984};
t878 = ct{3985};
t880 = ct{3986};
t881 = ct{3987};
t882 = ct{3988};
t884 = ct{3989};
t885 = ct{3990};
t888 = ct{3991};
t891 = ct{3992};
t893 = ct{3993};
t894 = ct{3994};
t895 = ct{3995};
t899 = ct{3996};
t9 = ct{3997};
t90 = ct{3998};
t900 = ct{3999};
t902 = ct{4000};
t903 = ct{4001};
t905 = ct{4002};
t906 = ct{4003};
t907 = ct{4004};
t908 = ct{4005};
t909 = ct{4006};
t91 = ct{4007};
t910 = ct{4008};
t911 = ct{4009};
t912 = ct{4010};
t913 = ct{4011};
t914 = ct{4012};
t915 = ct{4013};
t916 = ct{4014};
t917 = ct{4015};
t919 = ct{4016};
t920 = ct{4017};
t921 = ct{4018};
t922 = ct{4019};
t923 = ct{4020};
t925 = ct{4021};
t926 = ct{4022};
t927 = ct{4023};
t928 = ct{4024};
t929 = ct{4025};
t930 = ct{4026};
t931 = ct{4027};
t932 = ct{4028};
t934 = ct{4029};
t935 = ct{4030};
t937 = ct{4031};
t940 = ct{4032};
t941 = ct{4033};
t942 = ct{4034};
t943 = ct{4035};
t944 = ct{4036};
t945 = ct{4037};
t946 = ct{4038};
t947 = ct{4039};
t949 = ct{4040};
t95 = ct{4041};
t950 = ct{4042};
t951 = ct{4043};
t952 = ct{4044};
t953 = ct{4045};
t954 = ct{4046};
t955 = ct{4047};
t957 = ct{4048};
t958 = ct{4049};
t961 = ct{4050};
t962 = ct{4051};
t964 = ct{4052};
t965 = ct{4053};
t968 = ct{4054};
t97 = ct{4055};
t970 = ct{4056};
t971 = ct{4057};
t972 = ct{4058};
t973 = ct{4059};
t974 = ct{4060};
t975 = ct{4061};
t976 = ct{4062};
t977 = ct{4063};
t982 = ct{4064};
t983 = ct{4065};
t984 = ct{4066};
t985 = ct{4067};
t986 = ct{4068};
t987 = ct{4069};
t988 = ct{4070};
t989 = ct{4071};
t99 = ct{4072};
t990 = ct{4073};
t991 = ct{4074};
t993 = ct{4075};
t994 = ct{4076};
t995 = ct{4077};
t998 = ct{4078};
t999 = ct{4079};
t3991 = -t3963;
t3992 = -t3962;
t3993 = -t3964;
t3998 = -t3986;
t3999 = -t3987;
t4072 = -t4049;
t4076 = -t4059;
t4077 = -t4060;
t4078 = -t4061;
t4088 = -t4067;
t4096 = -t4082;
t4101 = -t4090;
t4102 = -t4094;
t4104 = -t4095;
t4107 = -t4098;
t4121 = -t4110;
t4122 = -t4111;
t4131 = t4106.^2;
t4137 = -t4128;
t4138 = -t4130;
t4146 = -t4136;
t4156 = t4.*t4126;
t4157 = t5.*t4126;
t4158 = t8.*t4126;
t4159 = t9.*t4126;
t4167 = t8.*t4147;
t4168 = t8.*t4148;
t4172 = -t4148;
t4175 = t4.*t4139;
t4176 = t8.*t4139;
t4198 = t5.*t4149;
t4199 = t9.*t4149;
t4528 = t645+t1451;
t4706 = t642+t1490;
t4838 = t1239+t1527;
t4891 = -t4843;
t4892 = -t4844;
t4917 = -t4859;
t4958 = -t4890;
t4972 = -t4896;
t4977 = -t4898;
t4985 = -t4905;
t5025 = t8.*t4889;
t5033 = -t4959;
t5040 = t8.*t4896;
t5042 = -t4965;
t5043 = t44.*t4126;
t5044 = t45.*t4126;
t5049 = t46.*t4126;
t5050 = t4148.*(-1.33637579258949e-4);
t5070 = t44.*t4139;
t5145 = t45.*t4149;
t5155 = -t5079;
t5163 = t57.*t4126;
t5168 = t59.*t4126;
t5169 = t60.*t4126;
t5170 = -t5094;
t5178 = -t5103;
t5196 = -t5124;
t5212 = -t5137;
t5230 = -t5160;
t5231 = t4147.*(-1.744166498897461e-6);
t5232 = t4148.*(-4.00912737776847e-7);
t5234 = t74.*t4126;
t5241 = -t5173;
t5246 = t75.*t4126;
t5253 = t76.*t4126;
t5254 = t4148.*(-1.246862701090643e-6);
t5256 = t77.*t4126;
t5259 = t80.*t4126;
t5260 = t57.*t4139;
t5263 = t83.*t4126;
t5264 = t4147.*(-3.383302988283333e-6);
t5266 = t4148.*(-3.383302988283333e-6);
t5273 = -t5214;
t5282 = -t5225;
t5284 = t8.*t5162;
t5290 = -t5243;
t5301 = t60.*t4149;
t5307 = t77.*t4139;
t5309 = t111.*t4126;
t5311 = -t5276;
t5312 = -t5277;
t5313 = -t5278;
t5314 = t83.*t4149;
t5315 = t114.*t4126;
t5335 = t74.*t4149;
t5337 = t75.*t4149;
t5338 = -t5304;
t5340 = t76.*t4149;
t5342 = t126.*t4126;
t5343 = t128.*t4126;
t5345 = t111.*t4139;
t5350 = -t5329;
t5352 = -t5336;
t5354 = t8.*t5275;
t5371 = t128.*t4139;
t5377 = t4147.*1.40259855e-11;
t5379 = t4148.*1.40259855e-11;
t5380 = t139.*t4126;
t5381 = t140.*t4126;
t5382 = t4147.*(-3.146556677756745e-13);
t5384 = t141.*t4126;
t5385 = t4148.*(-3.146556677756745e-13);
t5405 = t139.*t4139;
t5412 = t140.*t4149;
t5414 = t150.*t4126;
t5415 = t4147.*(-4.126305279697715e-13);
t5418 = t153.*t4126;
t5419 = t154.*t4126;
t5421 = t150.*t4139;
t5432 = t154.*t4149;
t5458 = -t5437;
t5509 = -t5500;
t5511 = -t5505;
t5529 = -t5518;
t5530 = -t5520;
t5538 = -t5524;
t5539 = -t5525;
t5545 = -t5531;
t5560 = -t5554;
t5564 = -t5556;
t5575 = -t5570;
t5576 = -t5571;
t5577 = -t5572;
t5591 = -t5587;
t5592 = -t5588;
t5602 = -t5601;
t5605 = (t613.*t4149)./2.0;
t5630 = t646+t648+t1447;
t5632 = -t5631;
t5662 = t203+t2421+t2463;
t5675 = -t5670;
t5684 = t1235+t1515+t1553;
t5686 = t3718+t3788;
t5687 = t3712+t3791;
t5695 = -t3.*(t3719-t3788);
t5697 = -t7.*(t3719-t3788);
t5770 = t4119.*t4126.*2.0;
t5772 = t4119.*t4149.*2.0;
t5774 = t5636.*(t50-t53).*(-1.0./2.0);
t5784 = t643+t647+t1448+t1479;
t5786 = t693+t2660+t3334;
t5787 = t689+t2657+t3331;
t5795 = t2541+t5599;
t5808 = t4106.*t4120.*3.038581678643136e-64;
t5810 = t1459+t5664;
t5811 = t1465+t5665;
t5816 = -t4.*(t1458-t5665);
t5817 = -t8.*(t1458-t5665);
t5820 = t4.*t5815;
t5821 = t8.*t5815;
t5822 = t1173+t1202+t1562+t2270;
t5827 = t4106.*t4120.*4.121912899099809e-68;
t5828 = t4106.*t4120.*1.879526485671887e-68;
t5831 = t4106.*t4120.*8.081970098144003e-70;
t5832 = t4106.*t4120.*5.344156668414146e-72;
t5835 = t4106.*t4120.*7.671525497590686e-73;
t5837 = (t484.*t5781)./2.0;
t5842 = t4106.*t5504.*3.038581678643136e-64;
t5850 = t1507+t4145+t4195;
t5867 = -t4.*(t7.*(t3719-t3788)+(t3.*t34.*t191.*(t29-t30))./8.112963841460668e+31);
t5868 = -t5.*(t7.*(t3719-t3788)+(t3.*t34.*t191.*(t29-t30))./8.112963841460668e+31);
t5869 = -t8.*(t7.*(t3719-t3788)+(t3.*t34.*t191.*(t29-t30))./8.112963841460668e+31);
t5870 = -t9.*(t7.*(t3719-t3788)+(t3.*t34.*t191.*(t29-t30))./8.112963841460668e+31);
t5876 = t4.*(t7.*(t3719-t3788)+(t3.*t34.*t191.*(t29-t30))./8.112963841460668e+31);
t5882 = t4106.*t5504.*1.879526485671887e-68;
t5883 = t4106.*t5504.*4.121912899099809e-68;
t5888 = t4106.*t5504.*8.081970098144003e-70;
t5889 = t4106.*t5504.*5.344156668414146e-72;
t5892 = t4106.*t5504.*7.671525497590686e-73;
t5919 = -t5917;
t5935 = (t5085.*t5781)./2.0;
t5939 = t676+t697+t2595+t2664+t3310;
t5940 = t660+t694+t2616+t2661+t3307;
t5959 = -t5958;
t5960 = (t5590.*t5781)./2.0;
t6001 = -t5998;
t6002 = -t5999;
t6007 = (t4126.*t5894)./2.0;
t6015 = (t4149.*t5894)./2.0;
t6064 = (t5688.*t5778)./2.0;
t6112 = t668+t686+t2587+t2594+t3236+t3251;
t6352 = t213+t698+t822+t2511+t2665+t2763+t3312+t3360;
t6410 = t685+t688+t2582+t2586+t3208+t3252+t5778;
t6411 = t682+t687+t2581+t2585+t3234+t3272+t5781;
t6609 = t649+t1689+t1726+t3362+t3790+t3886+t4376+t4430+t5310+t5317;
t4222 = -t4168;
t4238 = -t4175;
t4735 = t641+t1502;
t4743 = t3.*t4706;
t4744 = t7.*t4706;
t5144 = t4175.*(-1.33637579258949e-4);
t5228 = t4157.*4.00912737776847e-7;
t5235 = t4158.*(-7.26350610236655e-5);
t5286 = t4159.*(-1.744166498897461e-6);
t5296 = t4157.*(-1.246862701090643e-6);
t5299 = t4158.*(-4.20092050615074e-6);
t5316 = t4159.*2.179051830709965e-7;
t5323 = t4168.*(-4.00912737776847e-7);
t5333 = t4198.*4.00912737776847e-7;
t5357 = t4158.*(-2.524706033578261e-9);
t5369 = t4175.*(-1.758766830582798e-8);
t5370 = t4199.*2.179051830709965e-7;
t5396 = t4157.*1.40259855e-11;
t5397 = -t5377;
t5398 = t4159.*1.40259855e-11;
t5399 = -t5379;
t5401 = t4156.*(-3.146556677756745e-13);
t5403 = t4158.*(-3.146556677756745e-13);
t5422 = t4198.*1.40259855e-11;
t5423 = t4199.*1.40259855e-11;
t5426 = t4167.*(-1.40259855e-11);
t5427 = t4168.*(-1.40259855e-11);
t5428 = t4159.*(-4.126305279697715e-13);
t5431 = t4175.*(-4.126305279697715e-13);
t5447 = t4199.*(-4.126305279697715e-13);
t5515 = t4131./6.582018229284824e+63;
t5615 = t633+t4176;
t5617 = t4131.*2.060956449549905e-68;
t5619 = t4131.*9.397632428359433e-69;
t5623 = t4131.*4.040985049072001e-70;
t5626 = t4131.*2.672078334207073e-72;
t5628 = t4131.*3.835762748795343e-73;
t5657 = t2422+t4156;
t5661 = t2446+t4158;
t5671 = -t5.*(t2421-t4158);
t5672 = -t9.*(t2421-t4158);
t5689 = t3788+t3859;
t5690 = t3711+t3919;
t5691 = t3.*t5687;
t5692 = t4.*t5686;
t5693 = t7.*t5687;
t5694 = t8.*t5686;
t5703 = -t45.*(t2421-t4158);
t5705 = -t47.*(t2421-t4158);
t5712 = -t58.*(t2421-t4158);
t5713 = -t60.*(t2421-t4158);
t5718 = t5.*(t2421-t4158).*(-4.00912737776847e-7);
t5719 = -t71.*(t2421-t4158);
t5720 = t5.*(t2421-t4158).*7.26350610236655e-5;
t5721 = -t74.*(t2421-t4158);
t5722 = -t75.*(t2421-t4158);
t5724 = -t76.*(t2421-t4158);
t5726 = -t83.*(t2421-t4158);
t5728 = -t84.*(t2421-t4158);
t5731 = t5.*(t2421-t4158).*1.744166498897461e-6;
t5732 = t9.*(t2421-t4158).*1.744166498897461e-6;
t5733 = t5.*(t2421-t4158).*1.246862701090643e-6;
t5736 = t9.*(t2421-t4158).*3.383302988283333e-6;
t5738 = t9.*(t2421-t4158).*(-2.179051830709965e-7);
t5747 = -t140.*(t2421-t4158);
t5749 = -t142.*(t2421-t4158);
t5751 = t5.*(t2421-t4158).*(-1.40259855e-11);
t5753 = t9.*(t2421-t4158).*(-1.40259855e-11);
t5754 = t9.*(t2421-t4158).*3.146556677756745e-13;
t5758 = -t154.*(t2421-t4158);
t5759 = t5.*(t2421-t4158).*1.40259855e-11;
t5760 = t9.*(t2421-t4158).*1.40259855e-11;
t5764 = -t151.*(t2421-t4158);
t5765 = t9.*(t2421-t4158).*4.126305279697715e-13;
t5768 = t5.*(t2421-t4158).*4.126305279697715e-13;
t5771 = -t5770;
t5773 = -t5772;
t5775 = t4159+t4167;
t5789 = t577.*(t2421-t4158).*(-1.0./2.0);
t5792 = (t577.*(t2421-t4158))./2.0;
t5793 = ((t81-t86).*(t2421-t4158))./2.0;
t5809 = -t5808;
t5813 = t5.*t5810;
t5814 = t9.*t5810;
t5824 = t1289+t1501+t1513+t1529;
t5829 = -t5827;
t5830 = -t5828;
t5833 = -t5831;
t5834 = -t5832;
t5836 = -t5835;
t5838 = -t5837;
t5843 = -t5842;
t5851 = t1525+t4144+t4174;
t5854 = t3158+t5697;
t5861 = t3184+t5695;
t5884 = -t5882;
t5885 = -t5883;
t5890 = -t5888;
t5891 = -t5889;
t5893 = -t5892;
t5895 = t4742.*(t2421-t4158).*(-1.0./2.0);
t5898 = t4.*t5850.*3.52553938621e-7;
t5903 = t1516+t2477+t2485+t3191;
t5918 = t4.*t4119.*t5784;
t5925 = t204+t2478+t5787;
t5927 = t600.*(t4148+t5.*(t2421-t4158)).*(-1.0./2.0);
t5928 = (t600.*(t4148+t5.*(t2421-t4158)))./2.0;
t5931 = t4966.*t5784;
t5933 = t5086.*t5784;
t5936 = -t5935;
t5938 = t1460.*(t4148+t5.*(t2421-t4158)).*(-1.0./2.0);
t5954 = t2096.*(t4148+t5.*(t2421-t4158)).*(-1.0./2.0);
t5956 = (t2096.*(t4148+t5.*(t2421-t4158)))./2.0;
t5971 = t3444.*(t4148+t5.*(t2421-t4158)).*(-1.0./2.0);
t5976 = t5743.*(t2421-t4158).*(-1.0./2.0);
t5977 = t3514.*(t4148+t5.*(t2421-t4158)).*(-1.0./2.0);
t5978 = (t5743.*(t2421-t4158))./2.0;
t5979 = t639+t1442+t5850;
t5980 = (t5633.*t5787)./2.0;
t5981 = (t5634.*t5786)./2.0;
t5988 = -t4.*t4119.*(t4148+t5.*(t2421-t4158));
t5994 = t4.*t4119.*(t4148+t5.*(t2421-t4158));
t5996 = (t5939.*(t95-t4.*t9.*1.33637579258949e-4))./2.0;
t6000 = -t4528.*(t4148+t5.*(t2421-t4158));
t6006 = -t5784.*(t2421-t4158);
t6011 = -t6007;
t6012 = t5780.*(t2421-t4158).*(-1.0./2.0);
t6013 = t5784.*(t2421-t4158);
t6014 = (t5780.*(t2421-t4158))./2.0;
t6017 = -t6015;
t6031 = -t5086.*(t4148+t5.*(t2421-t4158));
t6060 = -t5406.*(t4148+t5.*(t2421-t4158));
t6061 = t4528.*(t4148+t5.*(t2421-t4158)).*(-7.26735e-3);
t6066 = t4528.*(t4148+t5.*(t2421-t4158)).*(-7.26350610236655e-5);
t6069 = t4528.*(t4148+t5.*(t2421-t4158)).*7.26350610236655e-5;
t6086 = t4528.*(t4148+t5.*(t2421-t4158)).*(-1.40259855e-11);
t6098 = t5669+t5817;
t6099 = t5675+t5816;
t6100 = t5673+t5821;
t6103 = t5678+t5820;
t6123 = -t5630.*(t4148+t5.*(t2421-t4158));
t6126 = t5630.*(t4148+t5.*(t2421-t4158));
t6136 = t205+t2467+t5940;
t6195 = (t4148+t5.*(t2421-t4158)).*(t2421-t4158);
t6203 = t5887.*(t2421-t4158).*(-1.0./2.0);
t6204 = (t5887.*(t2421-t4158))./2.0;
t6205 = (t5294.*t5939)./2.0;
t6206 = (t5321.*t5940)./2.0;
t6209 = (t5358.*t5939)./2.0;
t6210 = (t5361.*t5940)./2.0;
t6319 = -t5784.*(t4148+t5.*(t2421-t4158));
t6329 = (t5633.*t5939)./2.0;
t6330 = (t5634.*t5940)./2.0;
t6337 = t5784.*(t4148+t5.*(t2421-t4158)).*(-1.33637579258949e-4);
t6338 = t5784.*(t4148+t5.*(t2421-t4158)).*(-7.26735e-3);
t6341 = t5784.*(t4148+t5.*(t2421-t4158)).*1.33637579258949e-4;
t6342 = t5784.*(t4148+t5.*(t2421-t4158)).*7.26735e-3;
t6343 = t5784.*(t4148+t5.*(t2421-t4158)).*(-7.26350610236655e-5);
t6347 = t5784.*(t4148+t5.*(t2421-t4158)).*(-1.40259855e-11);
t6348 = t5784.*(t4148+t5.*(t2421-t4158)).*1.40259855e-11;
t6349 = t217+t702+t772+t2500+t2517+t2719+t2728+t3356;
t6350 = t210+t703+t775+t2520+t2536+t2685+t2731+t3357;
t6351 = t211+t696+t774+t2510+t2663+t2730+t3308+t3384;
t6362 = t5.*t6352.*7.01299275e-12;
t6391 = t661+t667+t1455+t1512+t1576+t4162+t4171+t4220;
t6395 = t665+t677+t1452+t1510+t1546+t4169+t4180+t4275;
t6403 = (t5688.*t6112)./2.0;
t6416 = t747+t763+t2622+t2648+t3286+t3327+t5786;
t6417 = t744+t759+t2620+t2644+t3320+t3326+t5787;
t6436 = t663+t675+t713+t756+t2603+t2608+t2629+t2679+t3282+t3325;
t6437 = t662+t674+t762+t815+t2602+t2607+t2647+t2670+t3287+t3295;
t6462 = t209+t695+t735+t776+t2503+t2535+t2662+t2678+t2732+t3335+t3358;
t6463 = t214+t728+t736+t782+t2512+t2522+t2682+t2699+t2735+t3313+t3359;
t6471 = (t5085.*t6411)./2.0;
t6506 = (t5590.*t6411)./2.0;
t6565 = (t5688.*t6410)./2.0;
t6597 = t657+t1631+t3346+t3692+t4362+t5044+t5169+t5190+t5226;
t6689 = t664+t700+t755+t768+t2590+t2604+t2613+t2628+t3280+t3299+t5939;
t6690 = t673+t683+t748+t764+t2606+t2623+t2639+t2649+t3277+t3296+t5940;
t6826 = t715+t758+t786+t795+t805+t837+t2631+t2636+t2680+t2701+t2705+t2746+t3290+t3301+t3342+t3374;
t6827 = t704+t711+t734+t751+t840+t888+t2626+t2668+t2676+t2677+t2712+t2738+t3289+t3297+t3350+t3367;
t7012 = t1580+t1599+t1698+t1830+t3403+t3405+t3630+t3697+t3797+t3948+t4310+t4415+t5315+t5342;
t7020 = t757+t769+t806+t921+t2614+t2630+t2729+t2747+t3283+t3302+t3341+t3354+t6352;
t7043 = t653+t1271+t1652+t2344+t2428+t3285+t3727+t3736+t4065+t4101+t4281+t4661+t4704+t5253+t5263+t5287+t5334+t5359;
t7079 = t1532+t1610+t1749+t1810+t2321+t2363+t2384+t2407+t2434+t2457+t3566+t3603+t3616+t3683+t4022+t4035+t4039+t4048+t4077+t4081+t4188+t4244+t4646+t4676+t4710+t4713;
t7080 = t1682+t1722+t1911+t2082+t2322+t2348+t2365+t2378+t2437+t2458+t3687+t3716+t3782+t3879+t4019+t4040+t4054+t4066+t4078+t4084+t4258+t4398+t4649+t4671+t4712+t4716;
t7087 = t692+t876+t894+t913+t920+t943+t951+t974+t990+t1107+t1277+t3333+t3347+t3382+t3431+t3448+t3456+t3466+t3467+t3470+t3487+t3494+t3497+t3509+t3529+t3533+t3549+t3586+t3599+t3730+t3774;
t7104 = t684+t729+t781+t792+t802+t826+t832+t875+t893+t912+t914+t1087+t1200+t3273+t3338+t3343+t3375+t3388+t3391+t3392+t3400+t3422+t3435+t3437+t3440+t3446+t3458+t3474+t3484+t3491+t3538+t3546+t3609+t3663;
t7119 = t1596+t1737+t1746+t1801+t1914+t2005+t2059+t2065+t2086+t2111+t2117+t2221+t3564+t3677+t3684+t3707+t3744+t3760+t3786+t3825+t3881+t3911+t3912+t3975+t4207+t4225+t4302+t4328+t4331+t4336+t4386+t4525;
t7256 = t710+t754+t798+t817+t829+t831+t848+t853+t902+t907+t916+t928+t931+t944+t953+t975+t976+t991+t1036+t1089+t1122+t1148+t1156+t1194+t1292+t1441+t3339+t3376+t3386+t3394+t3395+t3412+t3416+t3429+t3433+t3464+t3465+t3469+t3488+t3498+t3501+t3503+t3510+t3516+t3521+t3530+t3540+t3552+t3554+t3560+t3571+t3574+t3578+t3605+t3607+t3637+t3660+t3666+t3694+t3726+t4004+t4011+t4015;
t7333 = t1598+t1756+t1761+t1797+t1829+t1882+t1916+t1925+t1967+t1999+t2003+t2070+t2106+t2142+t2149+t2189+t2217+t2256+t2257+t2304+t2443+t2483+t2497+t2544+t2886+t2997+t3562+t3634+t3642+t3656+t3673+t3725+t3746+t3765+t3821+t3845+t3851+t3884+t3889+t3907+t3923+t3944+t3954+t3959+t3971+t3997+t4113+t4118+t4121+t4138+t4197+t4223+t4251+t4261+t4263+t4293+t4306+t4339+t4380+t4445+t4448+t4453+t4471+t4479+t4483+t4570+t4638+t4672+t4762+t4773;
t7364 = t680+t767+t794+t799+t848+t902+t928+t931+t944+t973+t975+t976+t991+t1122+t1156+t1194+t1292+t1441+t1817+t1988+t2029+t2056+t2094+t2175+t2204+t2251+t2302+t2487+t2518+t2527+t3365+t3404+t3416+t3424+t3429+t3449+t3464+t3465+t3469+t3498+t3501+t3510+t3521+t3530+t3540+t3554+t3571+t3574+t3578+t3587+t3605+t3607+t3637+t3665+t3666+t3694+t3726+t3830+t3864+t3900+t3916+t3936+t3961+t3988+t4004+t4009+t4011+t4015+t4109+t4129+t4135+t4316+t4372+t4422+t4455+t4532+t4535+t4554+t4603+t4615+t4765+t4774+t4776;
t7528 = t1551+t1627+t1648+t1710+t1742+t1848+t1855+t1908+t1929+t1954+t1986+t2018+t2045+t2057+t2062+t2101+t2123+t2125+t2135+t2143+t2181+t2187+t2196+t2202+t2213+t2237+t2258+t2289+t2312+t2332+t2346+t2371+t2392+t2426+t2473+t2530+t2539+t2542+t2554+t2556+t2560+t2627+t2822+t2839+t2852+t2904+t2914+t2917+t2931+t3000+t3015+t3220+t3237+t3246+t4308+t4357+t4379+t4411+t4413+t4461+t4466+t4469+t4477+t4493+t4497+t4520+t4529+t4551+t4559+t4564+t4567+t4573+t4581+t4584+t4590+t4591+t4594+t4605+t4607+t4610+t4614+t4618+t4620+t4622+t4631+t4635+t4655+t4667+t4669+t4689+t4693+t4694+t4697+t4702+t4715+t4724+t4730+t4732+t4745+t4755+t4757+t4768+t4784+t4786+t4787+t4857+t4951+t4991+t5005+t5015+t5036+t5073+t5089+t5146+t5172+t5183+t5187+t5191+t5209+t5224+t5240+t5295+t5306+t5435+t5440+t5441+t5453+t5473+t5475;
t7549 = t808+t814+t820+t885+t906+t927+t950+t961+t964+t983+t999+t1008+t1024+t1025+t1028+t1032+t1034+t1038+t1043+t1047+t1048+t1065+t1066+t1085+t1125+t1127+t1141+t1163+t1178+t1181+t1198+t1222+t1240+t1259+t1264+t1280+t1296+t1307+t1313+t1328+t1360+t1371+t1384+t1393+t1408+t1410+t1702+t1838+t1978+t2074+t2144+t2229+t2688+t2767+t2784+t2820+t2867+t2888+t2900+t2928+t2930+t2940+t2945+t2962+t2972+t2975+t2984+t2989+t2992+t3002+t3008+t3010+t3019+t3024+t3029+t3031+t3043+t3050+t3057+t3060+t3068+t3076+t3079+t3089+t3097+t3100+t3106+t3119+t3124+t3132+t3140+t3150+t3163+t3171+t3175+t3183+t3195+t3229+t3265+t3570+t3596+t3600+t3669+t3768+t3794+t3809+t3816+t3862+t3894+t3984+t3985+t4165+t4201+t4229+t4401+t4789+t4793+t4795+t4801+t4806+t4814+t4817+t4819+t4840+t4872+t4876+t4881+t4889+t4894+t4901+t4906+t4948+t4958+t4960+t4978+t5006+t5010+t5018+t5019+t5047+t5057+t5077+t5117+t5135+t5154+t5156+t5170+t5197+t5220+t5241+t5247+t5298+t5313+t5338+t5346+t5348+t5374+t5492+t5498+t5502+t5539;
t7553 = t1530+t1578+t1583+t1600+t1626+t1673+t1674+t1675+t1681+t1706+t1765+t1768+t1771+t1772+t1790+t1811+t1812+t1822+t1823+t1853+t1868+t1887+t1901+t1918+t1921+t1927+t1930+t1940+t1983+t1990+t1991+t1993+t2010+t2075+t2092+t2097+t2158+t2185+t2186+t2193+t2198+t2209+t2214+t2216+t2231+t2233+t2242+t2254+t2264+t2269+t2291+t2297+t2308+t2313+t2331+t2347+t2354+t2366+t2393+t2427+t2466+t2479+t2531+t2543+t2693+t2723+t2742+t2756+t2769+t2803+t2819+t2823+t2826+t2831+t2834+t2846+t2878+t2882+t2894+t2919+t2944+t2947+t2959+t2978+t3046+t3221+t3238+t3248+t4243+t4300+t4354+t4356+t4389+t4404+t4407+t4408+t4424+t4446+t4454+t4465+t4476+t4487+t4496+t4513+t4515+t4516+t4531+t4537+t4544+t4547+t4550+t4566+t4576+t4580+t4585+t4601+t4606+t4609+t4612+t4613+t4617+t4621+t4627+t4632+t4633+t4634+t4643+t4664+t4665+t4692+t4698+t4729+t4731+t4736+t4746+t4779+t4783+t4829+t4856+t4895+t4935+t4943+t4970+t4975+t5003+t5029+t5035+t5066+t5088+t5171+t5185+t5199+t5207+t5223+t5227+t5239+t5270+t5355+t5454+t5481+t5485;
t7556 = t882+t895+t900+t962+t977+t982+t995+t1013+t1044+t1051+t1055+t1059+t1093+t1102+t1109+t1115+t1116+t1130+t1138+t1153+t1167+t1175+t1183+t1197+t1210+t1219+t1244+t1251+t1302+t1309+t1312+t1319+t1326+t1341+t1346+t1355+t1362+t1366+t1374+t1375+t1385+t1389+t1397+t1406+t1415+t1433+t1463+t1464+t1478+t1481+t1774+t1976+t2129+t2157+t2274+t2318+t2489+t2540+t2869+t2892+t2908+t2920+t2923+t2969+t2980+t2985+t2991+t2996+t3007+t3014+t3027+t3030+t3033+t3048+t3053+t3055+t3059+t3070+t3072+t3073+t3074+t3086+t3090+t3112+t3118+t3121+t3127+t3128+t3130+t3131+t3146+t3152+t3153+t3157+t3167+t3174+t3178+t3180+t3187+t3190+t3196+t3232+t3254+t3269+t3291+t3293+t3323+t3423+t3461+t3595+t3631+t3740+t3778+t3855+t3861+t3877+t3888+t3946+t3989+t3994+t4006+t4098+t4105+t4125+t4142+t4242+t4321+t4375+t4740+t4790+t4791+t4794+t4812+t4813+t4823+t4835+t4844+t4859+t4863+t4874+t4893+t4931+t4939+t4965+t4976+t4985+t4992+t5014+t5037+t5041+t5054+t5079+t5095+t5103+t5124+t5126+t5134+t5137+t5138+t5141+t5158+t5180+t5230+t5272+t5277+t5282+t5288+t5303+t5330+t5350+t5351+t5352+t5365+t5388+t5437+t5448+t5460+t5500+t5524+t5531+t5587;
t7566 = t884+t891+t937+t942+t946+t949+t965+t987+t994+t1006+t1026+t1042+t1049+t1054+t1070+t1073+t1091+t1113+t1128+t1131+t1139+t1159+t1162+t1169+t1182+t1188+t1189+t1236+t1256+t1261+t1262+t1278+t1286+t1290+t1294+t1298+t1325+t1340+t1351+t1356+t1367+t1369+t1372+t1386+t1404+t1416+t1470+t1482+t1950+t1979+t2023+t2156+t2227+t2281+t2373+t2537+t2864+t2903+t2942+t2952+t2968+t2971+t2983+t2988+t3001+t3005+t3013+t3018+t3021+t3025+t3035+t3037+t3041+t3044+t3049+t3052+t3054+t3056+t3061+t3064+t3066+t3077+t3081+t3084+t3098+t3104+t3108+t3110+t3120+t3122+t3126+t3139+t3148+t3160+t3169+t3179+t3185+t3188+t3192+t3194+t3199+t3217+t3270+t3306+t3425+t3551+t3627+t3664+t3670+t3724+t3807+t3895+t3917+t3926+t3928+t3982+t4003+t4012+t4038+t4097+t4140+t4164+t4177+t4202+t4273+t4340+t4391+t4514+t4751+t4799+t4809+t4816+t4820+t4822+t4833+t4841+t4850+t4854+t4855+t4868+t4888+t4891+t4902+t4907+t4947+t4963+t4972+t4977+t5013+t5025+t5028+t5033+t5045+t5068+t5078+t5101+t5104+t5105+t5120+t5128+t5157+t5159+t5181+t5201+t5216+t5218+t5221+t5265+t5273+t5290+t5293+t5311+t5327+t5331+t5341+t5347+t5349+t5368+t5387+t5445+t5461+t5463+t5491+t5503+t5506+t5514+t5533+t5536+t5561+t5592;
t7570 = t1539+t1572+t1575+t1618+t1646+t1671+t1723+t1739+t1741+t1780+t1791+t1813+t1824+t1837+t1844+t1864+t1865+t1877+t1879+t1885+t1891+t1893+t1905+t1919+t1928+t1953+t1971+t1975+t1980+t1987+t2011+t2016+t2040+t2051+t2054+t2061+t2071+t2078+t2089+t2090+t2095+t2099+t2107+t2127+t2137+t2138+t2146+t2152+t2155+t2159+t2166+t2169+t2170+t2174+t2190+t2201+t2215+t2232+t2238+t2240+t2241+t2246+t2247+t2248+t2249+t2263+t2268+t2271+t2272+t2273+t2278+t2283+t2286+t2288+t2290+t2295+t2307+t2310+t2311+t2319+t2327+t2337+t2345+t2355+t2367+t2370+t2374+t2382+t2386+t2404+t2408+t2425+t2448+t2508+t2526+t2534+t2547+t2654+t2765+t2766+t2774+t2777+t2809+t2829+t2836+t2842+t2844+t2885+t2897+t2909+t2910+t2949+t2950+t2986+t2994+t2995+t3022+t3092+t3114+t3189+t3240+t3267+t4797+t4805+t4818+t4834+t4853+t4908+t4933+t5051+t5109+t5119+t5420+t5433+t5489+t5490+t5493+t5494+t5495+t5499+t5501+t5511+t5513+t5516+t5517+t5519+t5523+t5528+t5529+t5530+t5537+t5540+t5541+t5542+t5543+t5544+t5546+t5548+t5549+t5550+t5551+t5552+t5553+t5555+t5560+t5562+t5563+t5564+t5565+t5566+t5567+t5568+t5569+t5573+t5575+t5576+t5577+t5578+t5580+t5581+t5583+t5584+t5585+t5589+t5593+t5595+t5596+t5603+t5604+t5607+t5608+t5609+t5610+t5612+t5613+t5614+t5618+t5629+t5632+t5635;
et1 = t923+t935+t941+t988+t993+t1023+t1030+t1040+t1045+t1057+t1068+t1084+t1092+t1098+t1105+t1119+t1126+t1134+t1180+t1186+t1190+t1192+t1199+t1204+t1206+t1257+t1263+t1266+t1272+t1295+t1308+t1315+t1329+t1338+t1343+t1352+t1354+t1370+t1378+t1392+t1394+t1401+t1403+t1414+t1417+t1431+t1453+t1456+t1476+t1483+t1597+t1703+t1738+t1871+t1881+t1910+t1944+t1966+t2001+t2024+t2058+t2093+t2109+t2172+t2219+t2228+t2282+t2306+t2460+t2484+t2495+t2505+t2521+t2533+t2830+t2845+t2863+t2925+t2929+t2937+t2951+t2966+t2967+t2970+t3003+t3011+t3020+t3032+t3034+t3036+t3038+t3051+t3062+t3067+t3069+t3071+t3082+t3085+t3094+t3099+t3103+t3105+t3109+t3113+t3123+t3133+t3143+t3149+t3154+t3156+t3170+t3172+t3176+t3182+t3186+t3193+t3198+t3207+t3250+t3271+t3292+t3322+t3324+t3427+t3460+t3597+t3628+t3675+t3695+t3709+t3745+t3798+t3808+t3817+t3850+t3897+t3899+t3909+t3918+t3925+t3927+t3952+t3953+t3958+t3966+t3974+t3983+t3999+t4013+t4107+t4112+t4114+t4116+t4124+t4133+t4137+t4151+t4253+t4291+t4384+t4400+t4442+t4451+t4481+t4524+t4599+t4750+t4753+t4771+t4788+t4792+t4800+t4802+t4827+t4845+t4848+t4858+t4873+t4875+t4880+t4892+t4905+t4913+t4917+t4928+t4932+t4961+t5042+t5048+t5055+t5059+t5067+t5118+t5133+t5155+t5160+t5174+t5178+t5196+t5212;
et2 = t5213+t5225+t5229+t5248+t5268+t5292+t5308+t5312+t5326+t5329+t5332+t5336+t5367+t5386+t5444+t5458+t5462+t5509+t5538+t5545+t5591;
t7573 = et1+et2;
t4764 = t3.*t4735;
t4767 = t7.*t4735;
t5410 = -t5398;
t5622 = t634+t4238;
t5624 = t5.*t5615;
t5625 = t9.*t5615;
t5637 = t47.*t5615;
t5639 = t58.*t5615;
t5640 = t76.*t5615;
t5641 = t84.*t5615;
t5642 = t71.*t5615;
t5643 = t72.*t5615;
t5644 = t75.*t5615;
t5648 = t112.*t5615;
t5649 = t142.*t5615;
t5653 = t151.*t5615;
t5666 = t5657.^2;
t5679 = t2151+t4744;
t5680 = t2230+t4743;
t5682 = (t2088-t4743).^2;
t5696 = t4.*t5690;
t5698 = t8.*t5690;
t5699 = (t597.*t5615)./2.0;
t5701 = t47.*t5657;
t5704 = t9.*t5657.*(-1.33637579258949e-4);
t5707 = t58.*t5657;
t5711 = t71.*t5657;
t5714 = t75.*t5657;
t5715 = t76.*t5657;
t5716 = t84.*t5657;
t5723 = t9.*t5657.*(-1.246862701090643e-6);
t5727 = t9.*t5657.*(-3.383302988283333e-6);
t5742 = t142.*t5657;
t5745 = t5.*t5657.*1.40259855e-11;
t5746 = t9.*t5657.*1.40259855e-11;
t5748 = t9.*t5657.*(-3.146556677756745e-13);
t5757 = t151.*t5657;
t5763 = t5.*t5657.*(-4.126305279697715e-13);
t5776 = t4157+t4222;
t5788 = (t583.*t5657)./2.0;
t5790 = (t597.*t5657)./2.0;
t5794 = -t5793;
t5797 = (t638.*t5657)./2.0;
t5844 = t3606.*t5657;
t5845 = (t3523.*t5657)./2.0;
t5846 = t3757.*t5657;
t5849 = (t1471.*t5775)./2.0;
t5852 = t3134+t5693;
t5853 = t3161+t5691;
t5859 = t4.*t4119.*t5657.*2.0;
t5860 = (t3136-t5691).^2;
t5862 = -t5.*(t3136-t5691);
t5863 = -t9.*(t3136-t5691);
t5871 = t5861.^2;
t5872 = t4147+t5672;
t5873 = t5.*t5861;
t5874 = t9.*t5861;
t5875 = t5.*t8.*(t3136-t5691);
t5877 = t4172+t5671;
t5881 = t4528.*t5657;
t5896 = (t4763.*t5657)./2.0;
t5899 = t8.*t5851.*3.52553938621e-7;
t5901 = t4.*t4119.*t5657.*2.67275158517898e-4;
t5902 = t4.*t4119.*t5657.*1.45270122047331e-4;
t5905 = t4.*t4119.*t5657.*8.40184101230148e-6;
t5906 = t4.*t4119.*t5657.*6.293113355513489e-13;
t5909 = t4.*t4119.*t5657.*8.252610559395431e-13;
t5920 = -t5918;
t5930 = t5630.*t5657;
t5932 = t5918.*7.26735e-3;
t5934 = t5918.*2.180205e-5;
t5955 = t5657.*(t2421-t4158).*-2.0;
t5957 = t5657.*(t2421-t4158).*2.0;
t5963 = t5657.*(t2421-t4158).*(-2.67275158517898e-4);
t5964 = t5657.*(t2421-t4158).*2.67275158517898e-4;
t5965 = t5657.*(t2421-t4158).*(-1.45270122047331e-4);
t5966 = t5657.*(t2421-t4158).*(-8.40184101230148e-6);
t5967 = t5657.*(t2421-t4158).*(-6.293113355513489e-13);
t5969 = t5657.*(t2421-t4158).*(-8.252610559395431e-13);
t5970 = t5657.*(t2421-t4158).*8.252610559395431e-13;
t5972 = (t5657.*t5741)./2.0;
t5982 = (t1426.*t5925)./2.0;
t5984 = t5657.*t5775;
t6003 = (t5657.*t5777)./2.0;
t6005 = t5657.*t5784;
t6036 = t5994.*(-1.744166498897461e-6);
t6038 = t5994.*7.26350610236655e-5;
t6039 = t5994.*(-1.246862701090643e-6);
t6043 = t5994.*1.744166498897461e-6;
t6045 = t5994.*1.246862701090643e-6;
t6046 = t5994.*(-2.179051830709965e-7);
t6047 = t5994.*2.179051830709965e-7;
t6058 = t5994.*(-1.40259855e-11);
t6062 = t5994.*1.40259855e-11;
t6065 = t5994.*4.126305279697715e-13;
t6070 = t6013.*(-1.33637579258949e-4);
t6071 = t6013.*(-7.26735e-3);
t6075 = t6013.*1.33637579258949e-4;
t6077 = t6013.*7.26735e-3;
t6079 = t6013.*(-7.26350610236655e-5);
t6101 = t5.*t6098;
t6102 = t9.*t6098;
t6105 = t5.*t6100;
t6106 = t9.*t6100;
t6108 = (t5979.*(t95-t4.*t9.*1.33637579258949e-4))./2.0;
t6109 = t5775.*t5784;
t6117 = t5795.*(t2088-t4743).*(-3.038581678643136e-64);
t6119 = (t1426.*t5979)./2.0;
t6124 = (t5615.*t5886)./2.0;
t6139 = t5795.*(t2088-t4743).*(-4.121912899099809e-68);
t6140 = t5795.*(t2088-t4743).*(-1.879526485671887e-68);
t6149 = t5795.*(t2088-t4743).*(-8.081970098144003e-70);
